simulink library "BatteryPack_192S3P"  (R2025a)
settings: Solver=VariableStepAuto  StartTime=0.0  StopTime=10.0  RelTol=1e-3
undefined symbols (not defined in the file or in its folder): battery_builder_rtmsupport, gcbh
libraries: BatteryPack_192S3P_lib x28, nesl_utility x1, coolingPlateThermal_lib x1, fl_lib x1
(part 3 of 3)

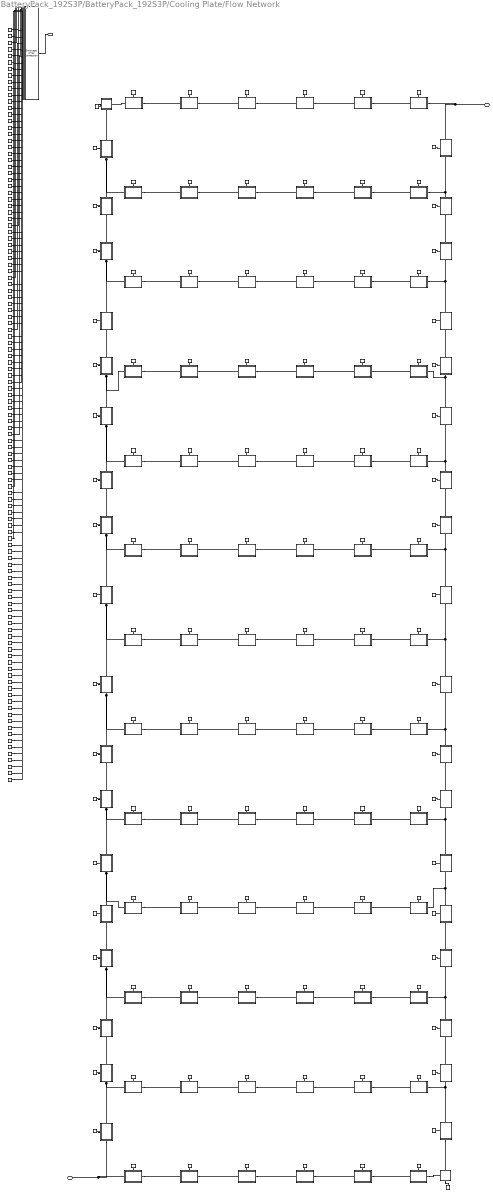
== system BatteryPack_192S3P/BatteryPack_192S3P/Cooling Plate/Flow Network ==
  note: Partition [6,8]
  note: Partition [6,7]
  note: Partition [6,6]
  note: Partition [6,5]
  note: Partition [6,4]
  note: Partition [6,3]
  note: Partition [6,2]
  note: Partition [6,1]
  note: Partition [5,8]
  note: Partition [5,7]
  note: Partition [5,6]
  note: Partition [5,5]
  note: Partition [5,4]
  note: Partition [5,3]
  note: Partition [5,2]
  note: Partition [5,1]
  note: Partition [4,8]
  note: Partition [4,7]
  note: Partition [4,6]
  note: Partition [4,5]
  note: Partition [4,4]
  note: Partition [4,3]
  note: Partition [4,2]
  note: Partition [4,1]
  note: Partition [3,8]
  note: Partition [3,7]
  note: Partition [3,6]
  note: Partition [3,5]
  note: Partition [3,4]
  note: Partition [3,3]
  note: Partition [3,2]
  note: Partition [3,1]
  note: Partition [2,8]
  note: Partition [2,7]
  note: Partition [2,6]
  note: Partition [2,5]
  note: Partition [2,4]
  note: Partition [2,3]
  note: Partition [2,2]
  note: Partition [2,1]
  note: Partition [1,8]
  note: Partition [1,7]
  note: Partition [1,6]
  note: Partition [1,5]
  note: Partition [1,4]
  note: Partition [1,3]
  note: Partition [1,2]
  note: Partition [1,1]
  Array Connection : SimscapeArrayConnection  Domain=foundation.thermal.thermal  NumScalarElements=116
  Bend1_1 : Subsystem  ReferencedSubsystem=BendSubsystemWithMask  lengthPipe=0.0031376  areaPipe=3.1416e-06  diaPipe=0.002  dirPipeOrientBend=up-right
      settings: PortSchema="{\"entries\":[{\"content\":{\"sides\":[{\"content\":{\"connectorIds\":[\"LConn1\"]},\"type\":\"ConnectorPlacement.EquallySpacedRectSide\",\"uuid\":\"064b9882-c01d-4ca6-b21a-bda87b570164\"},{\"content\":{\"side\":\"RIGHT\"},\"type\":\"ConnectorPlacement.EquallySpacedRectSide\",\"uuid\":\"eee751c1-0ee2-4a08-90dc-cac4f5822e04\"},{\"content\":{\"connectorIds\":[\"LConn2\"],\"side\":\"TOP\"},\"type\":\"ConnectorPlacement.EquallySpacedRectSide\",\"uuid\":\"508b7d1b-f548-4587-b0be-a567f0211289\"},{\"content\":{\"connectorIds\":[\"RConn1\"],\"side\":\"BOTTOM\"},\"type\":\"ConnectorPlacement.EquallySpacedRectSide\",\"uuid\":\"316bf1a6-1632-45cd-a339-45482f1cc5f7\"}]},\"type\":\"ConnectorPlacement.EquallySpacedConnector\",\"uuid\":\"7f420bea-eb7e-4a98-ba9c-58ec0a31ea83\"}],\"packageUris\":[\"http://schema.mathworks.com/mf0/Connector/R2020b\"],\"version\":\"1.0\"}"
  Bend2_1 : Subsystem  ReferencedSubsystem=BendSubsystemWithMask  lengthPipe=0.0031376  areaPipe=3.1416e-06  diaPipe=0.002  dirPipeOrientBend=up-right
      settings: PortSchema="{\"entries\":[{\"content\":{\"sides\":[{\"content\":{\"connectorIds\":[\"LConn1\"]},\"type\":\"ConnectorPlacement.EquallySpacedRectSide\",\"uuid\":\"064b9882-c01d-4ca6-b21a-bda87b570164\"},{\"content\":{\"side\":\"RIGHT\"},\"type\":\"ConnectorPlacement.EquallySpacedRectSide\",\"uuid\":\"eee751c1-0ee2-4a08-90dc-cac4f5822e04\"},{\"content\":{\"connectorIds\":[\"LConn2\"],\"side\":\"TOP\"},\"type\":\"ConnectorPlacement.EquallySpacedRectSide\",\"uuid\":\"508b7d1b-f548-4587-b0be-a567f0211289\"},{\"content\":{\"connectorIds\":[\"RConn1\"],\"side\":\"BOTTOM\"},\"type\":\"ConnectorPlacement.EquallySpacedRectSide\",\"uuid\":\"0f8d4577-782b-4a2e-bd78-882efcc560dd\"}]},\"type\":\"ConnectorPlacement.EquallySpacedConnector\",\"uuid\":\"7f420bea-eb7e-4a98-ba9c-58ec0a31ea83\"}],\"packageUris\":[\"http://schema.mathworks.com/mf0/Connector/R2020b\"],\"version\":\"1.0\"}"
  H_10_1 : ConnectionLabel  Label=H_10_1
  H_10_1_bus : ConnectionLabel  Label=H_10_1
  H_10_2 : ConnectionLabel  Label=H_10_2
  H_10_2_bus : ConnectionLabel  Label=H_10_2
  H_10_3 : ConnectionLabel  Label=H_10_3
  H_10_3_bus : ConnectionLabel  Label=H_10_3
  H_10_4 : ConnectionLabel  Label=H_10_4
  H_10_4_bus : ConnectionLabel  Label=H_10_4
  H_10_5 : ConnectionLabel  Label=H_10_5
  H_10_5_bus : ConnectionLabel  Label=H_10_5
  H_10_6 : ConnectionLabel  Label=H_10_6
  H_10_6_bus : ConnectionLabel  Label=H_10_6
  H_11_1 : ConnectionLabel  Label=H_11_1
  H_11_1_bus : ConnectionLabel  Label=H_11_1
  H_11_2 : ConnectionLabel  Label=H_11_2
  H_11_2_bus : ConnectionLabel  Label=H_11_2
  H_11_3 : ConnectionLabel  Label=H_11_3
  H_11_3_bus : ConnectionLabel  Label=H_11_3
  H_11_4 : ConnectionLabel  Label=H_11_4
  H_11_4_bus : ConnectionLabel  Label=H_11_4
  H_11_5 : ConnectionLabel  Label=H_11_5
  H_11_5_bus : ConnectionLabel  Label=H_11_5
  H_11_6 : ConnectionLabel  Label=H_11_6
  H_11_6_bus : ConnectionLabel  Label=H_11_6
  H_12_1 : ConnectionLabel  Label=H_12_1
  H_12_1_bus : ConnectionLabel  Label=H_12_1
  H_12_2 : ConnectionLabel  Label=H_12_2
  H_12_2_bus : ConnectionLabel  Label=H_12_2
  H_12_3 : ConnectionLabel  Label=H_12_3
  H_12_3_bus : ConnectionLabel  Label=H_12_3
  H_12_4 : ConnectionLabel  Label=H_12_4
  H_12_4_bus : ConnectionLabel  Label=H_12_4
  H_12_5 : ConnectionLabel  Label=H_12_5
  H_12_5_bus : ConnectionLabel  Label=H_12_5
  H_12_6 : ConnectionLabel  Label=H_12_6
  H_12_6_bus : ConnectionLabel  Label=H_12_6
  H_13_1 : ConnectionLabel  Label=H_13_1
  H_13_1_bus : ConnectionLabel  Label=H_13_1
  H_13_2 : ConnectionLabel  Label=H_13_2
  H_13_2_bus : ConnectionLabel  Label=H_13_2
  H_13_3 : ConnectionLabel  Label=H_13_3
  H_13_3_bus : ConnectionLabel  Label=H_13_3
  H_13_4 : ConnectionLabel  Label=H_13_4
  H_13_4_bus : ConnectionLabel  Label=H_13_4
  H_13_5 : ConnectionLabel  Label=H_13_5
  H_13_5_bus : ConnectionLabel  Label=H_13_5
  H_13_6 : ConnectionLabel  Label=H_13_6
  H_13_6_bus : ConnectionLabel  Label=H_13_6
  H_14_1 : ConnectionLabel  Label=H_14_1
  H_14_1_bus : ConnectionLabel  Label=H_14_1
  H_15_1 : ConnectionLabel  Label=H_15_1
  H_15_1_bus : ConnectionLabel  Label=H_15_1
  H_15_2 : ConnectionLabel  Label=H_15_2
  H_15_2_bus : ConnectionLabel  Label=H_15_2
  H_16_1 : ConnectionLabel  Label=H_16_1
  H_16_1_bus : ConnectionLabel  Label=H_16_1
  H_16_2 : ConnectionLabel  Label=H_16_2
  H_16_2_bus : ConnectionLabel  Label=H_16_2
  H_17_1 : ConnectionLabel  Label=H_17_1
  H_17_1_bus : ConnectionLabel  Label=H_17_1
  H_18_1 : ConnectionLabel  Label=H_18_1
  H_18_1_bus : ConnectionLabel  Label=H_18_1
  H_18_2 : ConnectionLabel  Label=H_18_2
  H_18_2_bus : ConnectionLabel  Label=H_18_2
  H_19_1 : ConnectionLabel  Label=H_19_1
  H_19_1_bus : ConnectionLabel  Label=H_19_1
  H_1_1 : ConnectionLabel  Label=H_1_1
  H_1_1_bus : ConnectionLabel  Label=H_1_1
  H_1_2 : ConnectionLabel  Label=H_1_2
  H_1_2_bus : ConnectionLabel  Label=H_1_2
  H_1_3 : ConnectionLabel  Label=H_1_3
  H_1_3_bus : ConnectionLabel  Label=H_1_3
  H_1_4 : ConnectionLabel  Label=H_1_4
  H_1_4_bus : ConnectionLabel  Label=H_1_4
  H_1_5 : ConnectionLabel  Label=H_1_5
  H_1_5_bus : ConnectionLabel  Label=H_1_5
  H_1_6 : ConnectionLabel  Label=H_1_6
  H_1_6_bus : ConnectionLabel  Label=H_1_6
  H_20_1 : ConnectionLabel  Label=H_20_1
  H_20_1_bus : ConnectionLabel  Label=H_20_1
  H_21_1 : ConnectionLabel  Label=H_21_1
  H_21_1_bus : ConnectionLabel  Label=H_21_1
  H_21_2 : ConnectionLabel  Label=H_21_2
  H_21_2_bus : ConnectionLabel  Label=H_21_2
  H_22_1 : ConnectionLabel  Label=H_22_1
  H_22_1_bus : ConnectionLabel  Label=H_22_1
  H_23_1 : ConnectionLabel  Label=H_23_1
  H_23_1_bus : ConnectionLabel  Label=H_23_1
  H_23_2 : ConnectionLabel  Label=H_23_2
  H_23_2_bus : ConnectionLabel  Label=H_23_2
  H_24_1 : ConnectionLabel  Label=H_24_1
  H_24_1_bus : ConnectionLabel  Label=H_24_1
  H_24_2 : ConnectionLabel  Label=H_24_2
  H_24_2_bus : ConnectionLabel  Label=H_24_2
  H_25_1 : ConnectionLabel  Label=H_25_1
  H_25_1_bus : ConnectionLabel  Label=H_25_1
  H_26_1 : ConnectionLabel  Label=H_26_1
  H_26_1_bus : ConnectionLabel  Label=H_26_1
  H_27_1 : ConnectionLabel  Label=H_27_1
  H_27_1_bus : ConnectionLabel  Label=H_27_1
  H_27_2 : ConnectionLabel  Label=H_27_2
  H_27_2_bus : ConnectionLabel  Label=H_27_2
  H_28_1 : ConnectionLabel  Label=H_28_1
  H_28_1_bus : ConnectionLabel  Label=H_28_1
  H_28_2 : ConnectionLabel  Label=H_28_2
  H_28_2_bus : ConnectionLabel  Label=H_28_2
  H_29_1 : ConnectionLabel  Label=H_29_1
  H_29_1_bus : ConnectionLabel  Label=H_29_1
  H_2_1 : ConnectionLabel  Label=H_2_1
  H_2_1_bus : ConnectionLabel  Label=H_2_1
  H_2_2 : ConnectionLabel  Label=H_2_2
  H_2_2_bus : ConnectionLabel  Label=H_2_2
  H_2_3 : ConnectionLabel  Label=H_2_3
  H_2_3_bus : ConnectionLabel  Label=H_2_3
  H_2_4 : ConnectionLabel  Label=H_2_4
  H_2_4_bus : ConnectionLabel  Label=H_2_4
  H_2_5 : ConnectionLabel  Label=H_2_5
  H_2_5_bus : ConnectionLabel  Label=H_2_5
  H_2_6 : ConnectionLabel  Label=H_2_6
  H_2_6_bus : ConnectionLabel  Label=H_2_6
  H_30_1 : ConnectionLabel  Label=H_30_1
  H_30_1_bus : ConnectionLabel  Label=H_30_1
  H_30_2 : ConnectionLabel  Label=H_30_2
  H_30_2_bus : ConnectionLabel  Label=H_30_2
  H_31_1 : ConnectionLabel  Label=H_31_1
  H_31_1_bus : ConnectionLabel  Label=H_31_1
  H_32_1 : ConnectionLabel  Label=H_32_1
  H_32_1_bus : ConnectionLabel  Label=H_32_1
  H_33_1 : ConnectionLabel  Label=H_33_1
  H_33_1_bus : ConnectionLabel  Label=H_33_1
  H_33_2 : ConnectionLabel  Label=H_33_2
  H_33_2_bus : ConnectionLabel  Label=H_33_2
  H_34_1 : ConnectionLabel  Label=H_34_1
  H_34_1_bus : ConnectionLabel  Label=H_34_1
  H_35_1 : ConnectionLabel  Label=H_35_1
  H_35_1_bus : ConnectionLabel  Label=H_35_1
  H_35_2 : ConnectionLabel  Label=H_35_2
  H_35_2_bus : ConnectionLabel  Label=H_35_2
  H_36_1 : ConnectionLabel  Label=H_36_1
  H_36_1_bus : ConnectionLabel  Label=H_36_1
  H_36_2 : ConnectionLabel  Label=H_36_2
  H_36_2_bus : ConnectionLabel  Label=H_36_2
  H_37_1 : ConnectionLabel  Label=H_37_1
  H_37_1_bus : ConnectionLabel  Label=H_37_1
  H_38_1 : ConnectionLabel  Label=H_38_1
  H_38_1_bus : ConnectionLabel  Label=H_38_1
  H_39_1 : ConnectionLabel  Label=H_39_1
  H_39_1_bus : ConnectionLabel  Label=H_39_1
  H_3_1 : ConnectionLabel  Label=H_3_1
  H_3_1_bus : ConnectionLabel  Label=H_3_1
  H_3_2 : ConnectionLabel  Label=H_3_2
  H_3_2_bus : ConnectionLabel  Label=H_3_2
  H_3_3 : ConnectionLabel  Label=H_3_3
  H_3_3_bus : ConnectionLabel  Label=H_3_3
  H_3_4 : ConnectionLabel  Label=H_3_4
  H_3_4_bus : ConnectionLabel  Label=H_3_4
  H_3_5 : ConnectionLabel  Label=H_3_5
  H_3_5_bus : ConnectionLabel  Label=H_3_5
  H_3_6 : ConnectionLabel  Label=H_3_6
  H_3_6_bus : ConnectionLabel  Label=H_3_6
  H_4_1 : ConnectionLabel  Label=H_4_1
  H_4_1_bus : ConnectionLabel  Label=H_4_1
  H_4_2 : ConnectionLabel  Label=H_4_2
  H_4_2_bus : ConnectionLabel  Label=H_4_2
  H_4_3 : ConnectionLabel  Label=H_4_3
  H_4_3_bus : ConnectionLabel  Label=H_4_3
  H_4_4 : ConnectionLabel  Label=H_4_4
  H_4_4_bus : ConnectionLabel  Label=H_4_4
  H_4_5 : ConnectionLabel  Label=H_4_5
  H_4_5_bus : ConnectionLabel  Label=H_4_5
  H_4_6 : ConnectionLabel  Label=H_4_6
  H_4_6_bus : ConnectionLabel  Label=H_4_6
  H_5_1 : ConnectionLabel  Label=H_5_1
  H_5_1_bus : ConnectionLabel  Label=H_5_1
  H_5_2 : ConnectionLabel  Label=H_5_2
  H_5_2_bus : ConnectionLabel  Label=H_5_2
  H_5_3 : ConnectionLabel  Label=H_5_3
  H_5_3_bus : ConnectionLabel  Label=H_5_3
  H_5_4 : ConnectionLabel  Label=H_5_4
  H_5_4_bus : ConnectionLabel  Label=H_5_4
  H_5_5 : ConnectionLabel  Label=H_5_5
  H_5_5_bus : ConnectionLabel  Label=H_5_5
  H_5_6 : ConnectionLabel  Label=H_5_6
  H_5_6_bus : ConnectionLabel  Label=H_5_6
  H_6_1 : ConnectionLabel  Label=H_6_1
  H_6_1_bus : ConnectionLabel  Label=H_6_1
  H_6_2 : ConnectionLabel  Label=H_6_2
  H_6_2_bus : ConnectionLabel  Label=H_6_2
  H_6_3 : ConnectionLabel  Label=H_6_3
  H_6_3_bus : ConnectionLabel  Label=H_6_3
  H_6_4 : ConnectionLabel  Label=H_6_4
  H_6_4_bus : ConnectionLabel  Label=H_6_4
  H_6_5 : ConnectionLabel  Label=H_6_5
  H_6_5_bus : ConnectionLabel  Label=H_6_5
  H_6_6 : ConnectionLabel  Label=H_6_6
  H_6_6_bus : ConnectionLabel  Label=H_6_6
  H_7_1 : ConnectionLabel  Label=H_7_1
  H_7_1_bus : ConnectionLabel  Label=H_7_1
  H_7_2 : ConnectionLabel  Label=H_7_2
  H_7_2_bus : ConnectionLabel  Label=H_7_2
  H_7_3 : ConnectionLabel  Label=H_7_3
  H_7_3_bus : ConnectionLabel  Label=H_7_3
  H_7_4 : ConnectionLabel  Label=H_7_4
  H_7_4_bus : ConnectionLabel  Label=H_7_4
  H_7_5 : ConnectionLabel  Label=H_7_5
  H_7_5_bus : ConnectionLabel  Label=H_7_5
  H_7_6 : ConnectionLabel  Label=H_7_6
  H_7_6_bus : ConnectionLabel  Label=H_7_6
  H_8_1 : ConnectionLabel  Label=H_8_1
  H_8_1_bus : ConnectionLabel  Label=H_8_1
  H_8_2 : ConnectionLabel  Label=H_8_2
  H_8_2_bus : ConnectionLabel  Label=H_8_2
  H_8_3 : ConnectionLabel  Label=H_8_3
  H_8_3_bus : ConnectionLabel  Label=H_8_3
  H_8_4 : ConnectionLabel  Label=H_8_4
  H_8_4_bus : ConnectionLabel  Label=H_8_4
  H_8_5 : ConnectionLabel  Label=H_8_5
  H_8_5_bus : ConnectionLabel  Label=H_8_5
  H_8_6 : ConnectionLabel  Label=H_8_6
  H_8_6_bus : ConnectionLabel  Label=H_8_6
  H_9_1 : ConnectionLabel  Label=H_9_1
  H_9_1_bus : ConnectionLabel  Label=H_9_1
  H_9_2 : ConnectionLabel  Label=H_9_2
  H_9_2_bus : ConnectionLabel  Label=H_9_2
  H_9_3 : ConnectionLabel  Label=H_9_3
  H_9_3_bus : ConnectionLabel  Label=H_9_3
  H_9_4 : ConnectionLabel  Label=H_9_4
  H_9_4_bus : ConnectionLabel  Label=H_9_4
  H_9_5 : ConnectionLabel  Label=H_9_5
  H_9_5_bus : ConnectionLabel  Label=H_9_5
  H_9_6 : ConnectionLabel  Label=H_9_6
  H_9_6_bus : ConnectionLabel  Label=H_9_6
  Pipe10_1 : Subsystem  ReferencedSubsystem=PipeSubsystemWithMask  lengthPipe=0.35833  areaPipe=3.1416e-06  diaPipe=0.002  directionPipe=right
      settings: PortSchema="{\"entries\":[{\"content\":{\"sides\":[{\"content\":{\"connectorIds\":[\"LConn1\"]},\"type\":\"ConnectorPlacement.EquallySpacedRectSide\",\"uuid\":\"064b9882-c01d-4ca6-b21a-bda87b570164\"},{\"content\":{\"connectorIds\":[\"RConn1\"],\"side\":\"RIGHT\"},\"type\":\"ConnectorPlacement.EquallySpacedRectSide\",\"uuid\":\"eee751c1-0ee2-4a08-90dc-cac4f5822e04\"},{\"content\":{\"connectorIds\":[\"LConn2\"],\"side\":\"TOP\"},\"type\":\"ConnectorPlacement.EquallySpacedRectSide\",\"uuid\":\"508b7d1b-f548-4587-b0be-a567f0211289\"}]},\"type\":\"ConnectorPlacement.EquallySpacedConnector\",\"uuid\":\"7f420bea-eb7e-4a98-ba9c-58ec0a31ea83\"}],\"packageUris\":[\"http://schema.mathworks.com/mf0/Connector/R2020b\"],\"version\":\"1.0\"}"
  Pipe10_{2..5} (4 alike) : Subsystem  ReferencedSubsystem=PipeSubsystemWithMask  lengthPipe=0.38333  areaPipe=3.1416e-06  diaPipe=0.002  directionPipe=right
      settings: PortSchema="{\"entries\":[{\"content\":{\"sides\":[{\"content\":{\"connectorIds\":[\"LConn1\"]},\"type\":\"ConnectorPlacement.EquallySpacedRectSide\",\"uuid\":\"064b9882-c01d-4ca6-b21a-bda87b570164\"},{\"content\":{\"connectorIds\":[\"RConn1\"],\"side\":\"RIGHT\"},\"type\":\"ConnectorPlacement.EquallySpacedRectSide\",\"uuid\":\"eee751c1-0ee2-4a08-90dc-cac4f5822e04\"},{\"content\":{\"connectorIds\":[\"LConn2\"],\"side\":\"TOP\"},\"type\":\"ConnectorPlacement.EquallySpacedRectSide\",\"uuid\":\"508b7d1b-f548-4587-b0be-a567f0211289\"}]},\"type\":\"ConnectorPlacement.EquallySpacedConnector\",\"uuid\":\"7f420bea-eb7e-4a98-ba9c-58ec0a31ea83\"}],\"packageUris\":[\"http://schema.mathworks.com/mf0/Connector/R2020b\"],\"version\":\"1.0\"}"
  Pipe10_6 : Subsystem  ReferencedSubsystem=PipeSubsystemWithMask  lengthPipe=0.35833  areaPipe=3.1416e-06  diaPipe=0.002  directionPipe=right
      settings: PortSchema="{\"entries\":[{\"content\":{\"sides\":[{\"content\":{\"connectorIds\":[\"LConn1\"]},\"type\":\"ConnectorPlacement.EquallySpacedRectSide\",\"uuid\":\"064b9882-c01d-4ca6-b21a-bda87b570164\"},{\"content\":{\"connectorIds\":[\"RConn1\"],\"side\":\"RIGHT\"},\"type\":\"ConnectorPlacement.EquallySpacedRectSide\",\"uuid\":\"eee751c1-0ee2-4a08-90dc-cac4f5822e04\"},{\"content\":{\"connectorIds\":[\"LConn2\"],\"side\":\"TOP\"},\"type\":\"ConnectorPlacement.EquallySpacedRectSide\",\"uuid\":\"508b7d1b-f548-4587-b0be-a567f0211289\"}]},\"type\":\"ConnectorPlacement.EquallySpacedConnector\",\"uuid\":\"7f420bea-eb7e-4a98-ba9c-58ec0a31ea83\"}],\"packageUris\":[\"http://schema.mathworks.com/mf0/Connector/R2020b\"],\"version\":\"1.0\"}"
  Pipe11_1 : Subsystem  ReferencedSubsystem=PipeSubsystemWithMask  lengthPipe=0.35833  areaPipe=3.1416e-06  diaPipe=0.002  directionPipe=right
      settings: PortSchema="{\"entries\":[{\"content\":{\"sides\":[{\"content\":{\"connectorIds\":[\"LConn1\"]},\"type\":\"ConnectorPlacement.EquallySpacedRectSide\",\"uuid\":\"064b9882-c01d-4ca6-b21a-bda87b570164\"},{\"content\":{\"connectorIds\":[\"RConn1\"],\"side\":\"RIGHT\"},\"type\":\"ConnectorPlacement.EquallySpacedRectSide\",\"uuid\":\"eee751c1-0ee2-4a08-90dc-cac4f5822e04\"},{\"content\":{\"connectorIds\":[\"LConn2\"],\"side\":\"TOP\"},\"type\":\"ConnectorPlacement.EquallySpacedRectSide\",\"uuid\":\"508b7d1b-f548-4587-b0be-a567f0211289\"}]},\"type\":\"ConnectorPlacement.EquallySpacedConnector\",\"uuid\":\"7f420bea-eb7e-4a98-ba9c-58ec0a31ea83\"}],\"packageUris\":[\"http://schema.mathworks.com/mf0/Connector/R2020b\"],\"version\":\"1.0\"}"
  Pipe11_{2..5} (4 alike) : Subsystem  ReferencedSubsystem=PipeSubsystemWithMask  lengthPipe=0.38333  areaPipe=3.1416e-06  diaPipe=0.002  directionPipe=right
      settings: PortSchema="{\"entries\":[{\"content\":{\"sides\":[{\"content\":{\"connectorIds\":[\"LConn1\"]},\"type\":\"ConnectorPlacement.EquallySpacedRectSide\",\"uuid\":\"064b9882-c01d-4ca6-b21a-bda87b570164\"},{\"content\":{\"connectorIds\":[\"RConn1\"],\"side\":\"RIGHT\"},\"type\":\"ConnectorPlacement.EquallySpacedRectSide\",\"uuid\":\"eee751c1-0ee2-4a08-90dc-cac4f5822e04\"},{\"content\":{\"connectorIds\":[\"LConn2\"],\"side\":\"TOP\"},\"type\":\"ConnectorPlacement.EquallySpacedRectSide\",\"uuid\":\"508b7d1b-f548-4587-b0be-a567f0211289\"}]},\"type\":\"ConnectorPlacement.EquallySpacedConnector\",\"uuid\":\"7f420bea-eb7e-4a98-ba9c-58ec0a31ea83\"}],\"packageUris\":[\"http://schema.mathworks.com/mf0/Connector/R2020b\"],\"version\":\"1.0\"}"
  Pipe11_6 : Subsystem  ReferencedSubsystem=PipeSubsystemWithMask  lengthPipe=0.35833  areaPipe=3.1416e-06  diaPipe=0.002  directionPipe=right
      settings: PortSchema="{\"entries\":[{\"content\":{\"sides\":[{\"content\":{\"connectorIds\":[\"LConn1\"]},\"type\":\"ConnectorPlacement.EquallySpacedRectSide\",\"uuid\":\"064b9882-c01d-4ca6-b21a-bda87b570164\"},{\"content\":{\"connectorIds\":[\"RConn1\"],\"side\":\"RIGHT\"},\"type\":\"ConnectorPlacement.EquallySpacedRectSide\",\"uuid\":\"eee751c1-0ee2-4a08-90dc-cac4f5822e04\"},{\"content\":{\"connectorIds\":[\"LConn2\"],\"side\":\"TOP\"},\"type\":\"ConnectorPlacement.EquallySpacedRectSide\",\"uuid\":\"508b7d1b-f548-4587-b0be-a567f0211289\"}]},\"type\":\"ConnectorPlacement.EquallySpacedConnector\",\"uuid\":\"7f420bea-eb7e-4a98-ba9c-58ec0a31ea83\"}],\"packageUris\":[\"http://schema.mathworks.com/mf0/Connector/R2020b\"],\"version\":\"1.0\"}"
  Pipe12_1 : Subsystem  ReferencedSubsystem=PipeSubsystemWithMask  lengthPipe=0.35833  areaPipe=3.1416e-06  diaPipe=0.002  directionPipe=right
      settings: PortSchema="{\"entries\":[{\"content\":{\"sides\":[{\"content\":{\"connectorIds\":[\"LConn1\"]},\"type\":\"ConnectorPlacement.EquallySpacedRectSide\",\"uuid\":\"064b9882-c01d-4ca6-b21a-bda87b570164\"},{\"content\":{\"connectorIds\":[\"RConn1\"],\"side\":\"RIGHT\"},\"type\":\"ConnectorPlacement.EquallySpacedRectSide\",\"uuid\":\"eee751c1-0ee2-4a08-90dc-cac4f5822e04\"},{\"content\":{\"connectorIds\":[\"LConn2\"],\"side\":\"TOP\"},\"type\":\"ConnectorPlacement.EquallySpacedRectSide\",\"uuid\":\"508b7d1b-f548-4587-b0be-a567f0211289\"}]},\"type\":\"ConnectorPlacement.EquallySpacedConnector\",\"uuid\":\"7f420bea-eb7e-4a98-ba9c-58ec0a31ea83\"}],\"packageUris\":[\"http://schema.mathworks.com/mf0/Connector/R2020b\"],\"version\":\"1.0\"}"
  Pipe12_{2..5} (4 alike) : Subsystem  ReferencedSubsystem=PipeSubsystemWithMask  lengthPipe=0.38333  areaPipe=3.1416e-06  diaPipe=0.002  directionPipe=right
      settings: PortSchema="{\"entries\":[{\"content\":{\"sides\":[{\"content\":{\"connectorIds\":[\"LConn1\"]},\"type\":\"ConnectorPlacement.EquallySpacedRectSide\",\"uuid\":\"064b9882-c01d-4ca6-b21a-bda87b570164\"},{\"content\":{\"connectorIds\":[\"RConn1\"],\"side\":\"RIGHT\"},\"type\":\"ConnectorPlacement.EquallySpacedRectSide\",\"uuid\":\"eee751c1-0ee2-4a08-90dc-cac4f5822e04\"},{\"content\":{\"connectorIds\":[\"LConn2\"],\"side\":\"TOP\"},\"type\":\"ConnectorPlacement.EquallySpacedRectSide\",\"uuid\":\"508b7d1b-f548-4587-b0be-a567f0211289\"}]},\"type\":\"ConnectorPlacement.EquallySpacedConnector\",\"uuid\":\"7f420bea-eb7e-4a98-ba9c-58ec0a31ea83\"}],\"packageUris\":[\"http://schema.mathworks.com/mf0/Connector/R2020b\"],\"version\":\"1.0\"}"
  Pipe12_6 : Subsystem  ReferencedSubsystem=PipeSubsystemWithMask  lengthPipe=0.35833  areaPipe=3.1416e-06  diaPipe=0.002  directionPipe=right
      settings: PortSchema="{\"entries\":[{\"content\":{\"sides\":[{\"content\":{\"connectorIds\":[\"LConn1\"]},\"type\":\"ConnectorPlacement.EquallySpacedRectSide\",\"uuid\":\"064b9882-c01d-4ca6-b21a-bda87b570164\"},{\"content\":{\"connectorIds\":[\"RConn1\"],\"side\":\"RIGHT\"},\"type\":\"ConnectorPlacement.EquallySpacedRectSide\",\"uuid\":\"eee751c1-0ee2-4a08-90dc-cac4f5822e04\"},{\"content\":{\"connectorIds\":[\"LConn2\"],\"side\":\"TOP\"},\"type\":\"ConnectorPlacement.EquallySpacedRectSide\",\"uuid\":\"508b7d1b-f548-4587-b0be-a567f0211289\"}]},\"type\":\"ConnectorPlacement.EquallySpacedConnector\",\"uuid\":\"7f420bea-eb7e-4a98-ba9c-58ec0a31ea83\"}],\"packageUris\":[\"http://schema.mathworks.com/mf0/Connector/R2020b\"],\"version\":\"1.0\"}"
  Pipe13_1 : Subsystem  ReferencedSubsystem=PipeSubsystemWithMask  lengthPipe=0.35633  areaPipe=3.1416e-06  diaPipe=0.002  directionPipe=right
      settings: PortSchema="{\"entries\":[{\"content\":{\"sides\":[{\"content\":{\"connectorIds\":[\"LConn1\"]},\"type\":\"ConnectorPlacement.EquallySpacedRectSide\",\"uuid\":\"064b9882-c01d-4ca6-b21a-bda87b570164\"},{\"content\":{\"connectorIds\":[\"RConn1\"],\"side\":\"RIGHT\"},\"type\":\"ConnectorPlacement.EquallySpacedRectSide\",\"uuid\":\"eee751c1-0ee2-4a08-90dc-cac4f5822e04\"},{\"content\":{\"connectorIds\":[\"LConn2\"],\"side\":\"TOP\"},\"type\":\"ConnectorPlacement.EquallySpacedRectSide\",\"uuid\":\"508b7d1b-f548-4587-b0be-a567f0211289\"}]},\"type\":\"ConnectorPlacement.EquallySpacedConnector\",\"uuid\":\"7f420bea-eb7e-4a98-ba9c-58ec0a31ea83\"}],\"packageUris\":[\"http://schema.mathworks.com/mf0/Connector/R2020b\"],\"version\":\"1.0\"}"
  Pipe13_{2..5} (4 alike) : Subsystem  ReferencedSubsystem=PipeSubsystemWithMask  lengthPipe=0.38333  areaPipe=3.1416e-06  diaPipe=0.002  directionPipe=right
      settings: PortSchema="{\"entries\":[{\"content\":{\"sides\":[{\"content\":{\"connectorIds\":[\"LConn1\"]},\"type\":\"ConnectorPlacement.EquallySpacedRectSide\",\"uuid\":\"064b9882-c01d-4ca6-b21a-bda87b570164\"},{\"content\":{\"connectorIds\":[\"RConn1\"],\"side\":\"RIGHT\"},\"type\":\"ConnectorPlacement.EquallySpacedRectSide\",\"uuid\":\"eee751c1-0ee2-4a08-90dc-cac4f5822e04\"},{\"content\":{\"connectorIds\":[\"LConn2\"],\"side\":\"TOP\"},\"type\":\"ConnectorPlacement.EquallySpacedRectSide\",\"uuid\":\"508b7d1b-f548-4587-b0be-a567f0211289\"}]},\"type\":\"ConnectorPlacement.EquallySpacedConnector\",\"uuid\":\"7f420bea-eb7e-4a98-ba9c-58ec0a31ea83\"}],\"packageUris\":[\"http://schema.mathworks.com/mf0/Connector/R2020b\"],\"version\":\"1.0\"}"
  Pipe13_6 : Subsystem  ReferencedSubsystem=PipeSubsystemWithMask  lengthPipe=0.35833  areaPipe=3.1416e-06  diaPipe=0.002  directionPipe=right
      settings: PortSchema="{\"entries\":[{\"content\":{\"sides\":[{\"content\":{\"connectorIds\":[\"LConn1\"]},\"type\":\"ConnectorPlacement.EquallySpacedRectSide\",\"uuid\":\"064b9882-c01d-4ca6-b21a-bda87b570164\"},{\"content\":{\"connectorIds\":[\"RConn1\"],\"side\":\"RIGHT\"},\"type\":\"ConnectorPlacement.EquallySpacedRectSide\",\"uuid\":\"eee751c1-0ee2-4a08-90dc-cac4f5822e04\"},{\"content\":{\"connectorIds\":[\"LConn2\"],\"side\":\"TOP\"},\"type\":\"ConnectorPlacement.EquallySpacedRectSide\",\"uuid\":\"508b7d1b-f548-4587-b0be-a567f0211289\"}]},\"type\":\"ConnectorPlacement.EquallySpacedConnector\",\"uuid\":\"7f420bea-eb7e-4a98-ba9c-58ec0a31ea83\"}],\"packageUris\":[\"http://schema.mathworks.com/mf0/Connector/R2020b\"],\"version\":\"1.0\"}"
  Pipe14_1 : Subsystem  ReferencedSubsystem=PipeSubsystemWithMask  lengthPipe=0.1  areaPipe=3.1416e-06  diaPipe=0.002  directionPipe=up
      settings: PortSchema="{\"entries\":[{\"content\":{\"sides\":[{\"content\":{\"connectorIds\":[\"LConn1\"]},\"type\":\"ConnectorPlacement.EquallySpacedRectSide\",\"uuid\":\"064b9882-c01d-4ca6-b21a-bda87b570164\"},{\"content\":{\"connectorIds\":[\"RConn1\"],\"side\":\"RIGHT\"},\"type\":\"ConnectorPlacement.EquallySpacedRectSide\",\"uuid\":\"eee751c1-0ee2-4a08-90dc-cac4f5822e04\"},{\"content\":{\"connectorIds\":[\"LConn2\"],\"side\":\"TOP\"},\"type\":\"ConnectorPlacement.EquallySpacedRectSide\",\"uuid\":\"508b7d1b-f548-4587-b0be-a567f0211289\"}]},\"type\":\"ConnectorPlacement.EquallySpacedConnector\",\"uuid\":\"7f420bea-eb7e-4a98-ba9c-58ec0a31ea83\"}],\"packageUris\":[\"http://schema.mathworks.com/mf0/Connector/R2020b\"],\"version\":\"1.0\"}"
  Pipe15_1 : Subsystem  ReferencedSubsystem=PipeSubsystemWithMask  lengthPipe=0.03125  areaPipe=3.1416e-06  diaPipe=0.002  directionPipe=up
      settings: PortSchema="{\"entries\":[{\"content\":{\"sides\":[{\"content\":{\"connectorIds\":[\"LConn1\"]},\"type\":\"ConnectorPlacement.EquallySpacedRectSide\",\"uuid\":\"064b9882-c01d-4ca6-b21a-bda87b570164\"},{\"content\":{\"connectorIds\":[\"RConn1\"],\"side\":\"RIGHT\"},\"type\":\"ConnectorPlacement.EquallySpacedRectSide\",\"uuid\":\"eee751c1-0ee2-4a08-90dc-cac4f5822e04\"},{\"content\":{\"connectorIds\":[\"LConn2\"],\"side\":\"TOP\"},\"type\":\"ConnectorPlacement.EquallySpacedRectSide\",\"uuid\":\"508b7d1b-f548-4587-b0be-a567f0211289\"}]},\"type\":\"ConnectorPlacement.EquallySpacedConnector\",\"uuid\":\"7f420bea-eb7e-4a98-ba9c-58ec0a31ea83\"}],\"packageUris\":[\"http://schema.mathworks.com/mf0/Connector/R2020b\"],\"version\":\"1.0\"}"
  Pipe15_2 : Subsystem  ReferencedSubsystem=PipeSubsystemWithMask  lengthPipe=0.06875  areaPipe=3.1416e-06  diaPipe=0.002  directionPipe=up
      settings: PortSchema="{\"entries\":[{\"content\":{\"sides\":[{\"content\":{\"connectorIds\":[\"LConn1\"]},\"type\":\"ConnectorPlacement.EquallySpacedRectSide\",\"uuid\":\"064b9882-c01d-4ca6-b21a-bda87b570164\"},{\"content\":{\"connectorIds\":[\"RConn1\"],\"side\":\"RIGHT\"},\"type\":\"ConnectorPlacement.EquallySpacedRectSide\",\"uuid\":\"eee751c1-0ee2-4a08-90dc-cac4f5822e04\"},{\"content\":{\"connectorIds\":[\"LConn2\"],\"side\":\"TOP\"},\"type\":\"ConnectorPlacement.EquallySpacedRectSide\",\"uuid\":\"508b7d1b-f548-4587-b0be-a567f0211289\"}]},\"type\":\"ConnectorPlacement.EquallySpacedConnector\",\"uuid\":\"7f420bea-eb7e-4a98-ba9c-58ec0a31ea83\"}],\"packageUris\":[\"http://schema.mathworks.com/mf0/Connector/R2020b\"],\"version\":\"1.0\"}"
  Pipe16_1 : Subsystem  ReferencedSubsystem=PipeSubsystemWithMask  lengthPipe=0.0875  areaPipe=3.1416e-06  diaPipe=0.002  directionPipe=up
      settings: PortSchema="{\"entries\":[{\"content\":{\"sides\":[{\"content\":{\"connectorIds\":[\"LConn1\"]},\"type\":\"ConnectorPlacement.EquallySpacedRectSide\",\"uuid\":\"064b9882-c01d-4ca6-b21a-bda87b570164\"},{\"content\":{\"connectorIds\":[\"RConn1\"],\"side\":\"RIGHT\"},\"type\":\"ConnectorPlacement.EquallySpacedRectSide\",\"uuid\":\"eee751c1-0ee2-4a08-90dc-cac4f5822e04\"},{\"content\":{\"connectorIds\":[\"LConn2\"],\"side\":\"TOP\"},\"type\":\"ConnectorPlacement.EquallySpacedRectSide\",\"uuid\":\"508b7d1b-f548-4587-b0be-a567f0211289\"}]},\"type\":\"ConnectorPlacement.EquallySpacedConnector\",\"uuid\":\"7f420bea-eb7e-4a98-ba9c-58ec0a31ea83\"}],\"packageUris\":[\"http://schema.mathworks.com/mf0/Connector/R2020b\"],\"version\":\"1.0\"}"
  Pipe16_2 : Subsystem  ReferencedSubsystem=PipeSubsystemWithMask  lengthPipe=0.0125  areaPipe=3.1416e-06  diaPipe=0.002  directionPipe=up
      settings: PortSchema="{\"entries\":[{\"content\":{\"sides\":[{\"content\":{\"connectorIds\":[\"LConn1\"]},\"type\":\"ConnectorPlacement.EquallySpacedRectSide\",\"uuid\":\"064b9882-c01d-4ca6-b21a-bda87b570164\"},{\"content\":{\"connectorIds\":[\"RConn1\"],\"side\":\"RIGHT\"},\"type\":\"ConnectorPlacement.EquallySpacedRectSide\",\"uuid\":\"eee751c1-0ee2-4a08-90dc-cac4f5822e04\"},{\"content\":{\"connectorIds\":[\"LConn2\"],\"side\":\"TOP\"},\"type\":\"ConnectorPlacement.EquallySpacedRectSide\",\"uuid\":\"508b7d1b-f548-4587-b0be-a567f0211289\"}]},\"type\":\"ConnectorPlacement.EquallySpacedConnector\",\"uuid\":\"7f420bea-eb7e-4a98-ba9c-58ec0a31ea83\"}],\"packageUris\":[\"http://schema.mathworks.com/mf0/Connector/R2020b\"],\"version\":\"1.0\"}"
  Pipe17_1 : Subsystem  ReferencedSubsystem=PipeSubsystemWithMask  lengthPipe=0.1  areaPipe=3.1416e-06  diaPipe=0.002  directionPipe=up
      settings: PortSchema="{\"entries\":[{\"content\":{\"sides\":[{\"content\":{\"connectorIds\":[\"LConn1\"]},\"type\":\"ConnectorPlacement.EquallySpacedRectSide\",\"uuid\":\"064b9882-c01d-4ca6-b21a-bda87b570164\"},{\"content\":{\"connectorIds\":[\"RConn1\"],\"side\":\"RIGHT\"},\"type\":\"ConnectorPlacement.EquallySpacedRectSide\",\"uuid\":\"eee751c1-0ee2-4a08-90dc-cac4f5822e04\"},{\"content\":{\"connectorIds\":[\"LConn2\"],\"side\":\"TOP\"},\"type\":\"ConnectorPlacement.EquallySpacedRectSide\",\"uuid\":\"508b7d1b-f548-4587-b0be-a567f0211289\"}]},\"type\":\"ConnectorPlacement.EquallySpacedConnector\",\"uuid\":\"7f420bea-eb7e-4a98-ba9c-58ec0a31ea83\"}],\"packageUris\":[\"http://schema.mathworks.com/mf0/Connector/R2020b\"],\"version\":\"1.0\"}"
  Pipe18_1 : Subsystem  ReferencedSubsystem=PipeSubsystemWithMask  lengthPipe=0.04375  areaPipe=3.1416e-06  diaPipe=0.002  directionPipe=up
      settings: PortSchema="{\"entries\":[{\"content\":{\"sides\":[{\"content\":{\"connectorIds\":[\"LConn1\"]},\"type\":\"ConnectorPlacement.EquallySpacedRectSide\",\"uuid\":\"064b9882-c01d-4ca6-b21a-bda87b570164\"},{\"content\":{\"connectorIds\":[\"RConn1\"],\"side\":\"RIGHT\"},\"type\":\"ConnectorPlacement.EquallySpacedRectSide\",\"uuid\":\"eee751c1-0ee2-4a08-90dc-cac4f5822e04\"},{\"content\":{\"connectorIds\":[\"LConn2\"],\"side\":\"TOP\"},\"type\":\"ConnectorPlacement.EquallySpacedRectSide\",\"uuid\":\"508b7d1b-f548-4587-b0be-a567f0211289\"}]},\"type\":\"ConnectorPlacement.EquallySpacedConnector\",\"uuid\":\"7f420bea-eb7e-4a98-ba9c-58ec0a31ea83\"}],\"packageUris\":[\"http://schema.mathworks.com/mf0/Connector/R2020b\"],\"version\":\"1.0\"}"
  Pipe18_2 : Subsystem  ReferencedSubsystem=PipeSubsystemWithMask  lengthPipe=0.05625  areaPipe=3.1416e-06  diaPipe=0.002  directionPipe=up
      settings: PortSchema="{\"entries\":[{\"content\":{\"sides\":[{\"content\":{\"connectorIds\":[\"LConn1\"]},\"type\":\"ConnectorPlacement.EquallySpacedRectSide\",\"uuid\":\"064b9882-c01d-4ca6-b21a-bda87b570164\"},{\"content\":{\"connectorIds\":[\"RConn1\"],\"side\":\"RIGHT\"},\"type\":\"ConnectorPlacement.EquallySpacedRectSide\",\"uuid\":\"eee751c1-0ee2-4a08-90dc-cac4f5822e04\"},{\"content\":{\"connectorIds\":[\"LConn2\"],\"side\":\"TOP\"},\"type\":\"ConnectorPlacement.EquallySpacedRectSide\",\"uuid\":\"508b7d1b-f548-4587-b0be-a567f0211289\"}]},\"type\":\"ConnectorPlacement.EquallySpacedConnector\",\"uuid\":\"7f420bea-eb7e-4a98-ba9c-58ec0a31ea83\"}],\"packageUris\":[\"http://schema.mathworks.com/mf0/Connector/R2020b\"],\"version\":\"1.0\"}"
  Pipe19_1 : Subsystem  ReferencedSubsystem=PipeSubsystemWithMask  lengthPipe=0.1  areaPipe=3.1416e-06  diaPipe=0.002  directionPipe=up
      settings: PortSchema="{\"entries\":[{\"content\":{\"sides\":[{\"content\":{\"connectorIds\":[\"LConn1\"]},\"type\":\"ConnectorPlacement.EquallySpacedRectSide\",\"uuid\":\"064b9882-c01d-4ca6-b21a-bda87b570164\"},{\"content\":{\"connectorIds\":[\"RConn1\"],\"side\":\"RIGHT\"},\"type\":\"ConnectorPlacement.EquallySpacedRectSide\",\"uuid\":\"eee751c1-0ee2-4a08-90dc-cac4f5822e04\"},{\"content\":{\"connectorIds\":[\"LConn2\"],\"side\":\"TOP\"},\"type\":\"ConnectorPlacement.EquallySpacedRectSide\",\"uuid\":\"508b7d1b-f548-4587-b0be-a567f0211289\"}]},\"type\":\"ConnectorPlacement.EquallySpacedConnector\",\"uuid\":\"7f420bea-eb7e-4a98-ba9c-58ec0a31ea83\"}],\"packageUris\":[\"http://schema.mathworks.com/mf0/Connector/R2020b\"],\"version\":\"1.0\"}"
  Pipe1_1 : Subsystem  ReferencedSubsystem=PipeSubsystemWithMask  lengthPipe=0.35833  areaPipe=3.1416e-06  diaPipe=0.002  directionPipe=right
      settings: PortSchema="{\"entries\":[{\"content\":{\"sides\":[{\"content\":{\"connectorIds\":[\"LConn1\"]},\"type\":\"ConnectorPlacement.EquallySpacedRectSide\",\"uuid\":\"064b9882-c01d-4ca6-b21a-bda87b570164\"},{\"content\":{\"connectorIds\":[\"RConn1\"],\"side\":\"RIGHT\"},\"type\":\"ConnectorPlacement.EquallySpacedRectSide\",\"uuid\":\"eee751c1-0ee2-4a08-90dc-cac4f5822e04\"},{\"content\":{\"connectorIds\":[\"LConn2\"],\"side\":\"TOP\"},\"type\":\"ConnectorPlacement.EquallySpacedRectSide\",\"uuid\":\"508b7d1b-f548-4587-b0be-a567f0211289\"}]},\"type\":\"ConnectorPlacement.EquallySpacedConnector\",\"uuid\":\"7f420bea-eb7e-4a98-ba9c-58ec0a31ea83\"}],\"packageUris\":[\"http://schema.mathworks.com/mf0/Connector/R2020b\"],\"version\":\"1.0\"}"
  Pipe1_{2..5} (4 alike) : Subsystem  ReferencedSubsystem=PipeSubsystemWithMask  lengthPipe=0.38333  areaPipe=3.1416e-06  diaPipe=0.002  directionPipe=right
      settings: PortSchema="{\"entries\":[{\"content\":{\"sides\":[{\"content\":{\"connectorIds\":[\"LConn1\"]},\"type\":\"ConnectorPlacement.EquallySpacedRectSide\",\"uuid\":\"064b9882-c01d-4ca6-b21a-bda87b570164\"},{\"content\":{\"connectorIds\":[\"RConn1\"],\"side\":\"RIGHT\"},\"type\":\"ConnectorPlacement.EquallySpacedRectSide\",\"uuid\":\"eee751c1-0ee2-4a08-90dc-cac4f5822e04\"},{\"content\":{\"connectorIds\":[\"LConn2\"],\"side\":\"TOP\"},\"type\":\"ConnectorPlacement.EquallySpacedRectSide\",\"uuid\":\"508b7d1b-f548-4587-b0be-a567f0211289\"}]},\"type\":\"ConnectorPlacement.EquallySpacedConnector\",\"uuid\":\"7f420bea-eb7e-4a98-ba9c-58ec0a31ea83\"}],\"packageUris\":[\"http://schema.mathworks.com/mf0/Connector/R2020b\"],\"version\":\"1.0\"}"
  Pipe1_6 : Subsystem  ReferencedSubsystem=PipeSubsystemWithMask  lengthPipe=0.35633  areaPipe=3.1416e-06  diaPipe=0.002  directionPipe=right
      settings: PortSchema="{\"entries\":[{\"content\":{\"sides\":[{\"content\":{\"connectorIds\":[\"LConn1\"]},\"type\":\"ConnectorPlacement.EquallySpacedRectSide\",\"uuid\":\"064b9882-c01d-4ca6-b21a-bda87b570164\"},{\"content\":{\"connectorIds\":[\"RConn1\"],\"side\":\"RIGHT\"},\"type\":\"ConnectorPlacement.EquallySpacedRectSide\",\"uuid\":\"eee751c1-0ee2-4a08-90dc-cac4f5822e04\"},{\"content\":{\"connectorIds\":[\"LConn2\"],\"side\":\"TOP\"},\"type\":\"ConnectorPlacement.EquallySpacedRectSide\",\"uuid\":\"508b7d1b-f548-4587-b0be-a567f0211289\"}]},\"type\":\"ConnectorPlacement.EquallySpacedConnector\",\"uuid\":\"7f420bea-eb7e-4a98-ba9c-58ec0a31ea83\"}],\"packageUris\":[\"http://schema.mathworks.com/mf0/Connector/R2020b\"],\"version\":\"1.0\"}"
  Pipe20_1 : Subsystem  ReferencedSubsystem=PipeSubsystemWithMask  lengthPipe=0.1  areaPipe=3.1416e-06  diaPipe=0.002  directionPipe=up
      settings: PortSchema="{\"entries\":[{\"content\":{\"sides\":[{\"content\":{\"connectorIds\":[\"LConn1\"]},\"type\":\"ConnectorPlacement.EquallySpacedRectSide\",\"uuid\":\"064b9882-c01d-4ca6-b21a-bda87b570164\"},{\"content\":{\"connectorIds\":[\"RConn1\"],\"side\":\"RIGHT\"},\"type\":\"ConnectorPlacement.EquallySpacedRectSide\",\"uuid\":\"eee751c1-0ee2-4a08-90dc-cac4f5822e04\"},{\"content\":{\"connectorIds\":[\"LConn2\"],\"side\":\"TOP\"},\"type\":\"ConnectorPlacement.EquallySpacedRectSide\",\"uuid\":\"508b7d1b-f548-4587-b0be-a567f0211289\"}]},\"type\":\"ConnectorPlacement.EquallySpacedConnector\",\"uuid\":\"7f420bea-eb7e-4a98-ba9c-58ec0a31ea83\"}],\"packageUris\":[\"http://schema.mathworks.com/mf0/Connector/R2020b\"],\"version\":\"1.0\"}"
  Pipe21_1 : Subsystem  ReferencedSubsystem=PipeSubsystemWithMask  lengthPipe=0.05625  areaPipe=3.1416e-06  diaPipe=0.002  directionPipe=up
      settings: PortSchema="{\"entries\":[{\"content\":{\"sides\":[{\"content\":{\"connectorIds\":[\"LConn1\"]},\"type\":\"ConnectorPlacement.EquallySpacedRectSide\",\"uuid\":\"064b9882-c01d-4ca6-b21a-bda87b570164\"},{\"content\":{\"connectorIds\":[\"RConn1\"],\"side\":\"RIGHT\"},\"type\":\"ConnectorPlacement.EquallySpacedRectSide\",\"uuid\":\"eee751c1-0ee2-4a08-90dc-cac4f5822e04\"},{\"content\":{\"connectorIds\":[\"LConn2\"],\"side\":\"TOP\"},\"type\":\"ConnectorPlacement.EquallySpacedRectSide\",\"uuid\":\"508b7d1b-f548-4587-b0be-a567f0211289\"}]},\"type\":\"ConnectorPlacement.EquallySpacedConnector\",\"uuid\":\"7f420bea-eb7e-4a98-ba9c-58ec0a31ea83\"}],\"packageUris\":[\"http://schema.mathworks.com/mf0/Connector/R2020b\"],\"version\":\"1.0\"}"
  Pipe21_2 : Subsystem  ReferencedSubsystem=PipeSubsystemWithMask  lengthPipe=0.04375  areaPipe=3.1416e-06  diaPipe=0.002  directionPipe=up
      settings: PortSchema="{\"entries\":[{\"content\":{\"sides\":[{\"content\":{\"connectorIds\":[\"LConn1\"]},\"type\":\"ConnectorPlacement.EquallySpacedRectSide\",\"uuid\":\"064b9882-c01d-4ca6-b21a-bda87b570164\"},{\"content\":{\"connectorIds\":[\"RConn1\"],\"side\":\"RIGHT\"},\"type\":\"ConnectorPlacement.EquallySpacedRectSide\",\"uuid\":\"eee751c1-0ee2-4a08-90dc-cac4f5822e04\"},{\"content\":{\"connectorIds\":[\"LConn2\"],\"side\":\"TOP\"},\"type\":\"ConnectorPlacement.EquallySpacedRectSide\",\"uuid\":\"508b7d1b-f548-4587-b0be-a567f0211289\"}]},\"type\":\"ConnectorPlacement.EquallySpacedConnector\",\"uuid\":\"7f420bea-eb7e-4a98-ba9c-58ec0a31ea83\"}],\"packageUris\":[\"http://schema.mathworks.com/mf0/Connector/R2020b\"],\"version\":\"1.0\"}"
  Pipe22_1 : Subsystem  ReferencedSubsystem=PipeSubsystemWithMask  lengthPipe=0.1  areaPipe=3.1416e-06  diaPipe=0.002  directionPipe=up
      settings: PortSchema="{\"entries\":[{\"content\":{\"sides\":[{\"content\":{\"connectorIds\":[\"LConn1\"]},\"type\":\"ConnectorPlacement.EquallySpacedRectSide\",\"uuid\":\"064b9882-c01d-4ca6-b21a-bda87b570164\"},{\"content\":{\"connectorIds\":[\"RConn1\"],\"side\":\"RIGHT\"},\"type\":\"ConnectorPlacement.EquallySpacedRectSide\",\"uuid\":\"eee751c1-0ee2-4a08-90dc-cac4f5822e04\"},{\"content\":{\"connectorIds\":[\"LConn2\"],\"side\":\"TOP\"},\"type\":\"ConnectorPlacement.EquallySpacedRectSide\",\"uuid\":\"508b7d1b-f548-4587-b0be-a567f0211289\"}]},\"type\":\"ConnectorPlacement.EquallySpacedConnector\",\"uuid\":\"7f420bea-eb7e-4a98-ba9c-58ec0a31ea83\"}],\"packageUris\":[\"http://schema.mathworks.com/mf0/Connector/R2020b\"],\"version\":\"1.0\"}"
  Pipe23_1 : Subsystem  ReferencedSubsystem=PipeSubsystemWithMask  lengthPipe=0.0125  areaPipe=3.1416e-06  diaPipe=0.002  directionPipe=up
      settings: PortSchema="{\"entries\":[{\"content\":{\"sides\":[{\"content\":{\"connectorIds\":[\"LConn1\"]},\"type\":\"ConnectorPlacement.EquallySpacedRectSide\",\"uuid\":\"064b9882-c01d-4ca6-b21a-bda87b570164\"},{\"content\":{\"connectorIds\":[\"RConn1\"],\"side\":\"RIGHT\"},\"type\":\"ConnectorPlacement.EquallySpacedRectSide\",\"uuid\":\"eee751c1-0ee2-4a08-90dc-cac4f5822e04\"},{\"content\":{\"connectorIds\":[\"LConn2\"],\"side\":\"TOP\"},\"type\":\"ConnectorPlacement.EquallySpacedRectSide\",\"uuid\":\"508b7d1b-f548-4587-b0be-a567f0211289\"}]},\"type\":\"ConnectorPlacement.EquallySpacedConnector\",\"uuid\":\"7f420bea-eb7e-4a98-ba9c-58ec0a31ea83\"}],\"packageUris\":[\"http://schema.mathworks.com/mf0/Connector/R2020b\"],\"version\":\"1.0\"}"
  Pipe23_2 : Subsystem  ReferencedSubsystem=PipeSubsystemWithMask  lengthPipe=0.0875  areaPipe=3.1416e-06  diaPipe=0.002  directionPipe=up
      settings: PortSchema="{\"entries\":[{\"content\":{\"sides\":[{\"content\":{\"connectorIds\":[\"LConn1\"]},\"type\":\"ConnectorPlacement.EquallySpacedRectSide\",\"uuid\":\"064b9882-c01d-4ca6-b21a-bda87b570164\"},{\"content\":{\"connectorIds\":[\"RConn1\"],\"side\":\"RIGHT\"},\"type\":\"ConnectorPlacement.EquallySpacedRectSide\",\"uuid\":\"eee751c1-0ee2-4a08-90dc-cac4f5822e04\"},{\"content\":{\"connectorIds\":[\"LConn2\"],\"side\":\"TOP\"},\"type\":\"ConnectorPlacement.EquallySpacedRectSide\",\"uuid\":\"508b7d1b-f548-4587-b0be-a567f0211289\"}]},\"type\":\"ConnectorPlacement.EquallySpacedConnector\",\"uuid\":\"7f420bea-eb7e-4a98-ba9c-58ec0a31ea83\"}],\"packageUris\":[\"http://schema.mathworks.com/mf0/Connector/R2020b\"],\"version\":\"1.0\"}"
  Pipe24_1 : Subsystem  ReferencedSubsystem=PipeSubsystemWithMask  lengthPipe=0.06875  areaPipe=3.1416e-06  diaPipe=0.002  directionPipe=up
      settings: PortSchema="{\"entries\":[{\"content\":{\"sides\":[{\"content\":{\"connectorIds\":[\"LConn1\"]},\"type\":\"ConnectorPlacement.EquallySpacedRectSide\",\"uuid\":\"064b9882-c01d-4ca6-b21a-bda87b570164\"},{\"content\":{\"connectorIds\":[\"RConn1\"],\"side\":\"RIGHT\"},\"type\":\"ConnectorPlacement.EquallySpacedRectSide\",\"uuid\":\"eee751c1-0ee2-4a08-90dc-cac4f5822e04\"},{\"content\":{\"connectorIds\":[\"LConn2\"],\"side\":\"TOP\"},\"type\":\"ConnectorPlacement.EquallySpacedRectSide\",\"uuid\":\"508b7d1b-f548-4587-b0be-a567f0211289\"}]},\"type\":\"ConnectorPlacement.EquallySpacedConnector\",\"uuid\":\"7f420bea-eb7e-4a98-ba9c-58ec0a31ea83\"}],\"packageUris\":[\"http://schema.mathworks.com/mf0/Connector/R2020b\"],\"version\":\"1.0\"}"
  Pipe24_2 : Subsystem  ReferencedSubsystem=PipeSubsystemWithMask  lengthPipe=0.03125  areaPipe=3.1416e-06  diaPipe=0.002  directionPipe=up
      settings: PortSchema="{\"entries\":[{\"content\":{\"sides\":[{\"content\":{\"connectorIds\":[\"LConn1\"]},\"type\":\"ConnectorPlacement.EquallySpacedRectSide\",\"uuid\":\"064b9882-c01d-4ca6-b21a-bda87b570164\"},{\"content\":{\"connectorIds\":[\"RConn1\"],\"side\":\"RIGHT\"},\"type\":\"ConnectorPlacement.EquallySpacedRectSide\",\"uuid\":\"eee751c1-0ee2-4a08-90dc-cac4f5822e04\"},{\"content\":{\"connectorIds\":[\"LConn2\"],\"side\":\"TOP\"},\"type\":\"ConnectorPlacement.EquallySpacedRectSide\",\"uuid\":\"508b7d1b-f548-4587-b0be-a567f0211289\"}]},\"type\":\"ConnectorPlacement.EquallySpacedConnector\",\"uuid\":\"7f420bea-eb7e-4a98-ba9c-58ec0a31ea83\"}],\"packageUris\":[\"http://schema.mathworks.com/mf0/Connector/R2020b\"],\"version\":\"1.0\"}"
  Pipe25_1 : Subsystem  ReferencedSubsystem=PipeSubsystemWithMask  lengthPipe=0.098  areaPipe=3.1416e-06  diaPipe=0.002  directionPipe=up
      settings: PortSchema="{\"entries\":[{\"content\":{\"sides\":[{\"content\":{\"connectorIds\":[\"LConn1\"]},\"type\":\"ConnectorPlacement.EquallySpacedRectSide\",\"uuid\":\"064b9882-c01d-4ca6-b21a-bda87b570164\"},{\"content\":{\"connectorIds\":[\"RConn1\"],\"side\":\"RIGHT\"},\"type\":\"ConnectorPlacement.EquallySpacedRectSide\",\"uuid\":\"eee751c1-0ee2-4a08-90dc-cac4f5822e04\"},{\"content\":{\"connectorIds\":[\"LConn2\"],\"side\":\"TOP\"},\"type\":\"ConnectorPlacement.EquallySpacedRectSide\",\"uuid\":\"508b7d1b-f548-4587-b0be-a567f0211289\"}]},\"type\":\"ConnectorPlacement.EquallySpacedConnector\",\"uuid\":\"7f420bea-eb7e-4a98-ba9c-58ec0a31ea83\"}],\"packageUris\":[\"http://schema.mathworks.com/mf0/Connector/R2020b\"],\"version\":\"1.0\"}"
  Pipe26_1 : Subsystem  ReferencedSubsystem=PipeSubsystemWithMask  lengthPipe=0.098  areaPipe=3.1416e-06  diaPipe=0.002  directionPipe=up
      settings: PortSchema="{\"entries\":[{\"content\":{\"sides\":[{\"content\":{\"connectorIds\":[\"LConn1\"]},\"type\":\"ConnectorPlacement.EquallySpacedRectSide\",\"uuid\":\"064b9882-c01d-4ca6-b21a-bda87b570164\"},{\"content\":{\"connectorIds\":[\"RConn1\"],\"side\":\"RIGHT\"},\"type\":\"ConnectorPlacement.EquallySpacedRectSide\",\"uuid\":\"eee751c1-0ee2-4a08-90dc-cac4f5822e04\"},{\"content\":{\"connectorIds\":[\"LConn2\"],\"side\":\"TOP\"},\"type\":\"ConnectorPlacement.EquallySpacedRectSide\",\"uuid\":\"508b7d1b-f548-4587-b0be-a567f0211289\"}]},\"type\":\"ConnectorPlacement.EquallySpacedConnector\",\"uuid\":\"7f420bea-eb7e-4a98-ba9c-58ec0a31ea83\"}],\"packageUris\":[\"http://schema.mathworks.com/mf0/Connector/R2020b\"],\"version\":\"1.0\"}"
  Pipe27_1 : Subsystem  ReferencedSubsystem=PipeSubsystemWithMask  lengthPipe=0.03125  areaPipe=3.1416e-06  diaPipe=0.002  directionPipe=up
      settings: PortSchema="{\"entries\":[{\"content\":{\"sides\":[{\"content\":{\"connectorIds\":[\"LConn1\"]},\"type\":\"ConnectorPlacement.EquallySpacedRectSide\",\"uuid\":\"064b9882-c01d-4ca6-b21a-bda87b570164\"},{\"content\":{\"connectorIds\":[\"RConn1\"],\"side\":\"RIGHT\"},\"type\":\"ConnectorPlacement.EquallySpacedRectSide\",\"uuid\":\"eee751c1-0ee2-4a08-90dc-cac4f5822e04\"},{\"content\":{\"connectorIds\":[\"LConn2\"],\"side\":\"TOP\"},\"type\":\"ConnectorPlacement.EquallySpacedRectSide\",\"uuid\":\"508b7d1b-f548-4587-b0be-a567f0211289\"}]},\"type\":\"ConnectorPlacement.EquallySpacedConnector\",\"uuid\":\"7f420bea-eb7e-4a98-ba9c-58ec0a31ea83\"}],\"packageUris\":[\"http://schema.mathworks.com/mf0/Connector/R2020b\"],\"version\":\"1.0\"}"
  Pipe27_2 : Subsystem  ReferencedSubsystem=PipeSubsystemWithMask  lengthPipe=0.06875  areaPipe=3.1416e-06  diaPipe=0.002  directionPipe=up
      settings: PortSchema="{\"entries\":[{\"content\":{\"sides\":[{\"content\":{\"connectorIds\":[\"LConn1\"]},\"type\":\"ConnectorPlacement.EquallySpacedRectSide\",\"uuid\":\"064b9882-c01d-4ca6-b21a-bda87b570164\"},{\"content\":{\"connectorIds\":[\"RConn1\"],\"side\":\"RIGHT\"},\"type\":\"ConnectorPlacement.EquallySpacedRectSide\",\"uuid\":\"eee751c1-0ee2-4a08-90dc-cac4f5822e04\"},{\"content\":{\"connectorIds\":[\"LConn2\"],\"side\":\"TOP\"},\"type\":\"ConnectorPlacement.EquallySpacedRectSide\",\"uuid\":\"508b7d1b-f548-4587-b0be-a567f0211289\"}]},\"type\":\"ConnectorPlacement.EquallySpacedConnector\",\"uuid\":\"7f420bea-eb7e-4a98-ba9c-58ec0a31ea83\"}],\"packageUris\":[\"http://schema.mathworks.com/mf0/Connector/R2020b\"],\"version\":\"1.0\"}"
  Pipe28_1 : Subsystem  ReferencedSubsystem=PipeSubsystemWithMask  lengthPipe=0.0875  areaPipe=3.1416e-06  diaPipe=0.002  directionPipe=up
      settings: PortSchema="{\"entries\":[{\"content\":{\"sides\":[{\"content\":{\"connectorIds\":[\"LConn1\"]},\"type\":\"ConnectorPlacement.EquallySpacedRectSide\",\"uuid\":\"064b9882-c01d-4ca6-b21a-bda87b570164\"},{\"content\":{\"connectorIds\":[\"RConn1\"],\"side\":\"RIGHT\"},\"type\":\"ConnectorPlacement.EquallySpacedRectSide\",\"uuid\":\"eee751c1-0ee2-4a08-90dc-cac4f5822e04\"},{\"content\":{\"connectorIds\":[\"LConn2\"],\"side\":\"TOP\"},\"type\":\"ConnectorPlacement.EquallySpacedRectSide\",\"uuid\":\"508b7d1b-f548-4587-b0be-a567f0211289\"}]},\"type\":\"ConnectorPlacement.EquallySpacedConnector\",\"uuid\":\"7f420bea-eb7e-4a98-ba9c-58ec0a31ea83\"}],\"packageUris\":[\"http://schema.mathworks.com/mf0/Connector/R2020b\"],\"version\":\"1.0\"}"
  Pipe28_2 : Subsystem  ReferencedSubsystem=PipeSubsystemWithMask  lengthPipe=0.0125  areaPipe=3.1416e-06  diaPipe=0.002  directionPipe=up
      settings: PortSchema="{\"entries\":[{\"content\":{\"sides\":[{\"content\":{\"connectorIds\":[\"LConn1\"]},\"type\":\"ConnectorPlacement.EquallySpacedRectSide\",\"uuid\":\"064b9882-c01d-4ca6-b21a-bda87b570164\"},{\"content\":{\"connectorIds\":[\"RConn1\"],\"side\":\"RIGHT\"},\"type\":\"ConnectorPlacement.EquallySpacedRectSide\",\"uuid\":\"eee751c1-0ee2-4a08-90dc-cac4f5822e04\"},{\"content\":{\"connectorIds\":[\"LConn2\"],\"side\":\"TOP\"},\"type\":\"ConnectorPlacement.EquallySpacedRectSide\",\"uuid\":\"508b7d1b-f548-4587-b0be-a567f0211289\"}]},\"type\":\"ConnectorPlacement.EquallySpacedConnector\",\"uuid\":\"7f420bea-eb7e-4a98-ba9c-58ec0a31ea83\"}],\"packageUris\":[\"http://schema.mathworks.com/mf0/Connector/R2020b\"],\"version\":\"1.0\"}"
  Pipe29_1 : Subsystem  ReferencedSubsystem=PipeSubsystemWithMask  lengthPipe=0.1  areaPipe=3.1416e-06  diaPipe=0.002  directionPipe=up
      settings: PortSchema="{\"entries\":[{\"content\":{\"sides\":[{\"content\":{\"connectorIds\":[\"LConn1\"]},\"type\":\"ConnectorPlacement.EquallySpacedRectSide\",\"uuid\":\"064b9882-c01d-4ca6-b21a-bda87b570164\"},{\"content\":{\"connectorIds\":[\"RConn1\"],\"side\":\"RIGHT\"},\"type\":\"ConnectorPlacement.EquallySpacedRectSide\",\"uuid\":\"eee751c1-0ee2-4a08-90dc-cac4f5822e04\"},{\"content\":{\"connectorIds\":[\"LConn2\"],\"side\":\"TOP\"},\"type\":\"ConnectorPlacement.EquallySpacedRectSide\",\"uuid\":\"508b7d1b-f548-4587-b0be-a567f0211289\"}]},\"type\":\"ConnectorPlacement.EquallySpacedConnector\",\"uuid\":\"7f420bea-eb7e-4a98-ba9c-58ec0a31ea83\"}],\"packageUris\":[\"http://schema.mathworks.com/mf0/Connector/R2020b\"],\"version\":\"1.0\"}"
  Pipe2_1 : Subsystem  ReferencedSubsystem=PipeSubsystemWithMask  lengthPipe=0.35833  areaPipe=3.1416e-06  diaPipe=0.002  directionPipe=right
      settings: PortSchema="{\"entries\":[{\"content\":{\"sides\":[{\"content\":{\"connectorIds\":[\"LConn1\"]},\"type\":\"ConnectorPlacement.EquallySpacedRectSide\",\"uuid\":\"064b9882-c01d-4ca6-b21a-bda87b570164\"},{\"content\":{\"connectorIds\":[\"RConn1\"],\"side\":\"RIGHT\"},\"type\":\"ConnectorPlacement.EquallySpacedRectSide\",\"uuid\":\"eee751c1-0ee2-4a08-90dc-cac4f5822e04\"},{\"content\":{\"connectorIds\":[\"LConn2\"],\"side\":\"TOP\"},\"type\":\"ConnectorPlacement.EquallySpacedRectSide\",\"uuid\":\"508b7d1b-f548-4587-b0be-a567f0211289\"}]},\"type\":\"ConnectorPlacement.EquallySpacedConnector\",\"uuid\":\"7f420bea-eb7e-4a98-ba9c-58ec0a31ea83\"}],\"packageUris\":[\"http://schema.mathworks.com/mf0/Connector/R2020b\"],\"version\":\"1.0\"}"
  Pipe2_{2..5} (4 alike) : Subsystem  ReferencedSubsystem=PipeSubsystemWithMask  lengthPipe=0.38333  areaPipe=3.1416e-06  diaPipe=0.002  directionPipe=right
      settings: PortSchema="{\"entries\":[{\"content\":{\"sides\":[{\"content\":{\"connectorIds\":[\"LConn1\"]},\"type\":\"ConnectorPlacement.EquallySpacedRectSide\",\"uuid\":\"064b9882-c01d-4ca6-b21a-bda87b570164\"},{\"content\":{\"connectorIds\":[\"RConn1\"],\"side\":\"RIGHT\"},\"type\":\"ConnectorPlacement.EquallySpacedRectSide\",\"uuid\":\"eee751c1-0ee2-4a08-90dc-cac4f5822e04\"},{\"content\":{\"connectorIds\":[\"LConn2\"],\"side\":\"TOP\"},\"type\":\"ConnectorPlacement.EquallySpacedRectSide\",\"uuid\":\"508b7d1b-f548-4587-b0be-a567f0211289\"}]},\"type\":\"ConnectorPlacement.EquallySpacedConnector\",\"uuid\":\"7f420bea-eb7e-4a98-ba9c-58ec0a31ea83\"}],\"packageUris\":[\"http://schema.mathworks.com/mf0/Connector/R2020b\"],\"version\":\"1.0\"}"
  Pipe2_6 : Subsystem  ReferencedSubsystem=PipeSubsystemWithMask  lengthPipe=0.35833  areaPipe=3.1416e-06  diaPipe=0.002  directionPipe=right
      settings: PortSchema="{\"entries\":[{\"content\":{\"sides\":[{\"content\":{\"connectorIds\":[\"LConn1\"]},\"type\":\"ConnectorPlacement.EquallySpacedRectSide\",\"uuid\":\"064b9882-c01d-4ca6-b21a-bda87b570164\"},{\"content\":{\"connectorIds\":[\"RConn1\"],\"side\":\"RIGHT\"},\"type\":\"ConnectorPlacement.EquallySpacedRectSide\",\"uuid\":\"eee751c1-0ee2-4a08-90dc-cac4f5822e04\"},{\"content\":{\"connectorIds\":[\"LConn2\"],\"side\":\"TOP\"},\"type\":\"ConnectorPlacement.EquallySpacedRectSide\",\"uuid\":\"508b7d1b-f548-4587-b0be-a567f0211289\"}]},\"type\":\"ConnectorPlacement.EquallySpacedConnector\",\"uuid\":\"7f420bea-eb7e-4a98-ba9c-58ec0a31ea83\"}],\"packageUris\":[\"http://schema.mathworks.com/mf0/Connector/R2020b\"],\"version\":\"1.0\"}"
  Pipe30_1 : Subsystem  ReferencedSubsystem=PipeSubsystemWithMask  lengthPipe=0.04375  areaPipe=3.1416e-06  diaPipe=0.002  directionPipe=up
      settings: PortSchema="{\"entries\":[{\"content\":{\"sides\":[{\"content\":{\"connectorIds\":[\"LConn1\"]},\"type\":\"ConnectorPlacement.EquallySpacedRectSide\",\"uuid\":\"064b9882-c01d-4ca6-b21a-bda87b570164\"},{\"content\":{\"connectorIds\":[\"RConn1\"],\"side\":\"RIGHT\"},\"type\":\"ConnectorPlacement.EquallySpacedRectSide\",\"uuid\":\"eee751c1-0ee2-4a08-90dc-cac4f5822e04\"},{\"content\":{\"connectorIds\":[\"LConn2\"],\"side\":\"TOP\"},\"type\":\"ConnectorPlacement.EquallySpacedRectSide\",\"uuid\":\"508b7d1b-f548-4587-b0be-a567f0211289\"}]},\"type\":\"ConnectorPlacement.EquallySpacedConnector\",\"uuid\":\"7f420bea-eb7e-4a98-ba9c-58ec0a31ea83\"}],\"packageUris\":[\"http://schema.mathworks.com/mf0/Connector/R2020b\"],\"version\":\"1.0\"}"
  Pipe30_2 : Subsystem  ReferencedSubsystem=PipeSubsystemWithMask  lengthPipe=0.05625  areaPipe=3.1416e-06  diaPipe=0.002  directionPipe=up
      settings: PortSchema="{\"entries\":[{\"content\":{\"sides\":[{\"content\":{\"connectorIds\":[\"LConn1\"]},\"type\":\"ConnectorPlacement.EquallySpacedRectSide\",\"uuid\":\"064b9882-c01d-4ca6-b21a-bda87b570164\"},{\"content\":{\"connectorIds\":[\"RConn1\"],\"side\":\"RIGHT\"},\"type\":\"ConnectorPlacement.EquallySpacedRectSide\",\"uuid\":\"eee751c1-0ee2-4a08-90dc-cac4f5822e04\"},{\"content\":{\"connectorIds\":[\"LConn2\"],\"side\":\"TOP\"},\"type\":\"ConnectorPlacement.EquallySpacedRectSide\",\"uuid\":\"508b7d1b-f548-4587-b0be-a567f0211289\"}]},\"type\":\"ConnectorPlacement.EquallySpacedConnector\",\"uuid\":\"7f420bea-eb7e-4a98-ba9c-58ec0a31ea83\"}],\"packageUris\":[\"http://schema.mathworks.com/mf0/Connector/R2020b\"],\"version\":\"1.0\"}"
  Pipe31_1 : Subsystem  ReferencedSubsystem=PipeSubsystemWithMask  lengthPipe=0.1  areaPipe=3.1416e-06  diaPipe=0.002  directionPipe=up
      settings: PortSchema="{\"entries\":[{\"content\":{\"sides\":[{\"content\":{\"connectorIds\":[\"LConn1\"]},\"type\":\"ConnectorPlacement.EquallySpacedRectSide\",\"uuid\":\"064b9882-c01d-4ca6-b21a-bda87b570164\"},{\"content\":{\"connectorIds\":[\"RConn1\"],\"side\":\"RIGHT\"},\"type\":\"ConnectorPlacement.EquallySpacedRectSide\",\"uuid\":\"eee751c1-0ee2-4a08-90dc-cac4f5822e04\"},{\"content\":{\"connectorIds\":[\"LConn2\"],\"side\":\"TOP\"},\"type\":\"ConnectorPlacement.EquallySpacedRectSide\",\"uuid\":\"508b7d1b-f548-4587-b0be-a567f0211289\"}]},\"type\":\"ConnectorPlacement.EquallySpacedConnector\",\"uuid\":\"7f420bea-eb7e-4a98-ba9c-58ec0a31ea83\"}],\"packageUris\":[\"http://schema.mathworks.com/mf0/Connector/R2020b\"],\"version\":\"1.0\"}"
  Pipe32_1 : Subsystem  ReferencedSubsystem=PipeSubsystemWithMask  lengthPipe=0.1  areaPipe=3.1416e-06  diaPipe=0.002  directionPipe=up
      settings: PortSchema="{\"entries\":[{\"content\":{\"sides\":[{\"content\":{\"connectorIds\":[\"LConn1\"]},\"type\":\"ConnectorPlacement.EquallySpacedRectSide\",\"uuid\":\"064b9882-c01d-4ca6-b21a-bda87b570164\"},{\"content\":{\"connectorIds\":[\"RConn1\"],\"side\":\"RIGHT\"},\"type\":\"ConnectorPlacement.EquallySpacedRectSide\",\"uuid\":\"eee751c1-0ee2-4a08-90dc-cac4f5822e04\"},{\"content\":{\"connectorIds\":[\"LConn2\"],\"side\":\"TOP\"},\"type\":\"ConnectorPlacement.EquallySpacedRectSide\",\"uuid\":\"508b7d1b-f548-4587-b0be-a567f0211289\"}]},\"type\":\"ConnectorPlacement.EquallySpacedConnector\",\"uuid\":\"7f420bea-eb7e-4a98-ba9c-58ec0a31ea83\"}],\"packageUris\":[\"http://schema.mathworks.com/mf0/Connector/R2020b\"],\"version\":\"1.0\"}"
  Pipe33_1 : Subsystem  ReferencedSubsystem=PipeSubsystemWithMask  lengthPipe=0.05625  areaPipe=3.1416e-06  diaPipe=0.002  directionPipe=up
      settings: PortSchema="{\"entries\":[{\"content\":{\"sides\":[{\"content\":{\"connectorIds\":[\"LConn1\"]},\"type\":\"ConnectorPlacement.EquallySpacedRectSide\",\"uuid\":\"064b9882-c01d-4ca6-b21a-bda87b570164\"},{\"content\":{\"connectorIds\":[\"RConn1\"],\"side\":\"RIGHT\"},\"type\":\"ConnectorPlacement.EquallySpacedRectSide\",\"uuid\":\"eee751c1-0ee2-4a08-90dc-cac4f5822e04\"},{\"content\":{\"connectorIds\":[\"LConn2\"],\"side\":\"TOP\"},\"type\":\"ConnectorPlacement.EquallySpacedRectSide\",\"uuid\":\"508b7d1b-f548-4587-b0be-a567f0211289\"}]},\"type\":\"ConnectorPlacement.EquallySpacedConnector\",\"uuid\":\"7f420bea-eb7e-4a98-ba9c-58ec0a31ea83\"}],\"packageUris\":[\"http://schema.mathworks.com/mf0/Connector/R2020b\"],\"version\":\"1.0\"}"
  Pipe33_2 : Subsystem  ReferencedSubsystem=PipeSubsystemWithMask  lengthPipe=0.04375  areaPipe=3.1416e-06  diaPipe=0.002  directionPipe=up
      settings: PortSchema="{\"entries\":[{\"content\":{\"sides\":[{\"content\":{\"connectorIds\":[\"LConn1\"]},\"type\":\"ConnectorPlacement.EquallySpacedRectSide\",\"uuid\":\"064b9882-c01d-4ca6-b21a-bda87b570164\"},{\"content\":{\"connectorIds\":[\"RConn1\"],\"side\":\"RIGHT\"},\"type\":\"ConnectorPlacement.EquallySpacedRectSide\",\"uuid\":\"eee751c1-0ee2-4a08-90dc-cac4f5822e04\"},{\"content\":{\"connectorIds\":[\"LConn2\"],\"side\":\"TOP\"},\"type\":\"ConnectorPlacement.EquallySpacedRectSide\",\"uuid\":\"508b7d1b-f548-4587-b0be-a567f0211289\"}]},\"type\":\"ConnectorPlacement.EquallySpacedConnector\",\"uuid\":\"7f420bea-eb7e-4a98-ba9c-58ec0a31ea83\"}],\"packageUris\":[\"http://schema.mathworks.com/mf0/Connector/R2020b\"],\"version\":\"1.0\"}"
  Pipe34_1 : Subsystem  ReferencedSubsystem=PipeSubsystemWithMask  lengthPipe=0.1  areaPipe=3.1416e-06  diaPipe=0.002  directionPipe=up
      settings: PortSchema="{\"entries\":[{\"content\":{\"sides\":[{\"content\":{\"connectorIds\":[\"LConn1\"]},\"type\":\"ConnectorPlacement.EquallySpacedRectSide\",\"uuid\":\"064b9882-c01d-4ca6-b21a-bda87b570164\"},{\"content\":{\"connectorIds\":[\"RConn1\"],\"side\":\"RIGHT\"},\"type\":\"ConnectorPlacement.EquallySpacedRectSide\",\"uuid\":\"eee751c1-0ee2-4a08-90dc-cac4f5822e04\"},{\"content\":{\"connectorIds\":[\"LConn2\"],\"side\":\"TOP\"},\"type\":\"ConnectorPlacement.EquallySpacedRectSide\",\"uuid\":\"508b7d1b-f548-4587-b0be-a567f0211289\"}]},\"type\":\"ConnectorPlacement.EquallySpacedConnector\",\"uuid\":\"7f420bea-eb7e-4a98-ba9c-58ec0a31ea83\"}],\"packageUris\":[\"http://schema.mathworks.com/mf0/Connector/R2020b\"],\"version\":\"1.0\"}"
  Pipe35_1 : Subsystem  ReferencedSubsystem=PipeSubsystemWithMask  lengthPipe=0.0125  areaPipe=3.1416e-06  diaPipe=0.002  directionPipe=up
      settings: PortSchema="{\"entries\":[{\"content\":{\"sides\":[{\"content\":{\"connectorIds\":[\"LConn1\"]},\"type\":\"ConnectorPlacement.EquallySpacedRectSide\",\"uuid\":\"064b9882-c01d-4ca6-b21a-bda87b570164\"},{\"content\":{\"connectorIds\":[\"RConn1\"],\"side\":\"RIGHT\"},\"type\":\"ConnectorPlacement.EquallySpacedRectSide\",\"uuid\":\"eee751c1-0ee2-4a08-90dc-cac4f5822e04\"},{\"content\":{\"connectorIds\":[\"LConn2\"],\"side\":\"TOP\"},\"type\":\"ConnectorPlacement.EquallySpacedRectSide\",\"uuid\":\"508b7d1b-f548-4587-b0be-a567f0211289\"}]},\"type\":\"ConnectorPlacement.EquallySpacedConnector\",\"uuid\":\"7f420bea-eb7e-4a98-ba9c-58ec0a31ea83\"}],\"packageUris\":[\"http://schema.mathworks.com/mf0/Connector/R2020b\"],\"version\":\"1.0\"}"
  Pipe35_2 : Subsystem  ReferencedSubsystem=PipeSubsystemWithMask  lengthPipe=0.0875  areaPipe=3.1416e-06  diaPipe=0.002  directionPipe=up
      settings: PortSchema="{\"entries\":[{\"content\":{\"sides\":[{\"content\":{\"connectorIds\":[\"LConn1\"]},\"type\":\"ConnectorPlacement.EquallySpacedRectSide\",\"uuid\":\"064b9882-c01d-4ca6-b21a-bda87b570164\"},{\"content\":{\"connectorIds\":[\"RConn1\"],\"side\":\"RIGHT\"},\"type\":\"ConnectorPlacement.EquallySpacedRectSide\",\"uuid\":\"eee751c1-0ee2-4a08-90dc-cac4f5822e04\"},{\"content\":{\"connectorIds\":[\"LConn2\"],\"side\":\"TOP\"},\"type\":\"ConnectorPlacement.EquallySpacedRectSide\",\"uuid\":\"508b7d1b-f548-4587-b0be-a567f0211289\"}]},\"type\":\"ConnectorPlacement.EquallySpacedConnector\",\"uuid\":\"7f420bea-eb7e-4a98-ba9c-58ec0a31ea83\"}],\"packageUris\":[\"http://schema.mathworks.com/mf0/Connector/R2020b\"],\"version\":\"1.0\"}"
  Pipe36_1 : Subsystem  ReferencedSubsystem=PipeSubsystemWithMask  lengthPipe=0.06875  areaPipe=3.1416e-06  diaPipe=0.002  directionPipe=up
      settings: PortSchema="{\"entries\":[{\"content\":{\"sides\":[{\"content\":{\"connectorIds\":[\"LConn1\"]},\"type\":\"ConnectorPlacement.EquallySpacedRectSide\",\"uuid\":\"064b9882-c01d-4ca6-b21a-bda87b570164\"},{\"content\":{\"connectorIds\":[\"RConn1\"],\"side\":\"RIGHT\"},\"type\":\"ConnectorPlacement.EquallySpacedRectSide\",\"uuid\":\"eee751c1-0ee2-4a08-90dc-cac4f5822e04\"},{\"content\":{\"connectorIds\":[\"LConn2\"],\"side\":\"TOP\"},\"type\":\"ConnectorPlacement.EquallySpacedRectSide\",\"uuid\":\"508b7d1b-f548-4587-b0be-a567f0211289\"}]},\"type\":\"ConnectorPlacement.EquallySpacedConnector\",\"uuid\":\"7f420bea-eb7e-4a98-ba9c-58ec0a31ea83\"}],\"packageUris\":[\"http://schema.mathworks.com/mf0/Connector/R2020b\"],\"version\":\"1.0\"}"
  Pipe36_2 : Subsystem  ReferencedSubsystem=PipeSubsystemWithMask  lengthPipe=0.03125  areaPipe=3.1416e-06  diaPipe=0.002  directionPipe=up
      settings: PortSchema="{\"entries\":[{\"content\":{\"sides\":[{\"content\":{\"connectorIds\":[\"LConn1\"]},\"type\":\"ConnectorPlacement.EquallySpacedRectSide\",\"uuid\":\"064b9882-c01d-4ca6-b21a-bda87b570164\"},{\"content\":{\"connectorIds\":[\"RConn1\"],\"side\":\"RIGHT\"},\"type\":\"ConnectorPlacement.EquallySpacedRectSide\",\"uuid\":\"eee751c1-0ee2-4a08-90dc-cac4f5822e04\"},{\"content\":{\"connectorIds\":[\"LConn2\"],\"side\":\"TOP\"},\"type\":\"ConnectorPlacement.EquallySpacedRectSide\",\"uuid\":\"508b7d1b-f548-4587-b0be-a567f0211289\"}]},\"type\":\"ConnectorPlacement.EquallySpacedConnector\",\"uuid\":\"7f420bea-eb7e-4a98-ba9c-58ec0a31ea83\"}],\"packageUris\":[\"http://schema.mathworks.com/mf0/Connector/R2020b\"],\"version\":\"1.0\"}"
  Pipe37_1 : Subsystem  ReferencedSubsystem=PipeSubsystemWithMask  lengthPipe=0.1  areaPipe=3.1416e-06  diaPipe=0.002  directionPipe=up
      settings: PortSchema="{\"entries\":[{\"content\":{\"sides\":[{\"content\":{\"connectorIds\":[\"LConn1\"]},\"type\":\"ConnectorPlacement.EquallySpacedRectSide\",\"uuid\":\"064b9882-c01d-4ca6-b21a-bda87b570164\"},{\"content\":{\"connectorIds\":[\"RConn1\"],\"side\":\"RIGHT\"},\"type\":\"ConnectorPlacement.EquallySpacedRectSide\",\"uuid\":\"eee751c1-0ee2-4a08-90dc-cac4f5822e04\"},{\"content\":{\"connectorIds\":[\"LConn2\"],\"side\":\"TOP\"},\"type\":\"ConnectorPlacement.EquallySpacedRectSide\",\"uuid\":\"508b7d1b-f548-4587-b0be-a567f0211289\"}]},\"type\":\"ConnectorPlacement.EquallySpacedConnector\",\"uuid\":\"7f420bea-eb7e-4a98-ba9c-58ec0a31ea83\"}],\"packageUris\":[\"http://schema.mathworks.com/mf0/Connector/R2020b\"],\"version\":\"1.0\"}"
  Pipe3_1 : Subsystem  ReferencedSubsystem=PipeSubsystemWithMask  lengthPipe=0.35833  areaPipe=3.1416e-06  diaPipe=0.002  directionPipe=right
      settings: PortSchema="{\"entries\":[{\"content\":{\"sides\":[{\"content\":{\"connectorIds\":[\"LConn1\"]},\"type\":\"ConnectorPlacement.EquallySpacedRectSide\",\"uuid\":\"064b9882-c01d-4ca6-b21a-bda87b570164\"},{\"content\":{\"connectorIds\":[\"RConn1\"],\"side\":\"RIGHT\"},\"type\":\"ConnectorPlacement.EquallySpacedRectSide\",\"uuid\":\"eee751c1-0ee2-4a08-90dc-cac4f5822e04\"},{\"content\":{\"connectorIds\":[\"LConn2\"],\"side\":\"TOP\"},\"type\":\"ConnectorPlacement.EquallySpacedRectSide\",\"uuid\":\"508b7d1b-f548-4587-b0be-a567f0211289\"}]},\"type\":\"ConnectorPlacement.EquallySpacedConnector\",\"uuid\":\"7f420bea-eb7e-4a98-ba9c-58ec0a31ea83\"}],\"packageUris\":[\"http://schema.mathworks.com/mf0/Connector/R2020b\"],\"version\":\"1.0\"}"
  Pipe3_{2..5} (4 alike) : Subsystem  ReferencedSubsystem=PipeSubsystemWithMask  lengthPipe=0.38333  areaPipe=3.1416e-06  diaPipe=0.002  directionPipe=right
      settings: PortSchema="{\"entries\":[{\"content\":{\"sides\":[{\"content\":{\"connectorIds\":[\"LConn1\"]},\"type\":\"ConnectorPlacement.EquallySpacedRectSide\",\"uuid\":\"064b9882-c01d-4ca6-b21a-bda87b570164\"},{\"content\":{\"connectorIds\":[\"RConn1\"],\"side\":\"RIGHT\"},\"type\":\"ConnectorPlacement.EquallySpacedRectSide\",\"uuid\":\"eee751c1-0ee2-4a08-90dc-cac4f5822e04\"},{\"content\":{\"connectorIds\":[\"LConn2\"],\"side\":\"TOP\"},\"type\":\"ConnectorPlacement.EquallySpacedRectSide\",\"uuid\":\"508b7d1b-f548-4587-b0be-a567f0211289\"}]},\"type\":\"ConnectorPlacement.EquallySpacedConnector\",\"uuid\":\"7f420bea-eb7e-4a98-ba9c-58ec0a31ea83\"}],\"packageUris\":[\"http://schema.mathworks.com/mf0/Connector/R2020b\"],\"version\":\"1.0\"}"
  Pipe3_6 : Subsystem  ReferencedSubsystem=PipeSubsystemWithMask  lengthPipe=0.35833  areaPipe=3.1416e-06  diaPipe=0.002  directionPipe=right
      settings: PortSchema="{\"entries\":[{\"content\":{\"sides\":[{\"content\":{\"connectorIds\":[\"LConn1\"]},\"type\":\"ConnectorPlacement.EquallySpacedRectSide\",\"uuid\":\"064b9882-c01d-4ca6-b21a-bda87b570164\"},{\"content\":{\"connectorIds\":[\"RConn1\"],\"side\":\"RIGHT\"},\"type\":\"ConnectorPlacement.EquallySpacedRectSide\",\"uuid\":\"eee751c1-0ee2-4a08-90dc-cac4f5822e04\"},{\"content\":{\"connectorIds\":[\"LConn2\"],\"side\":\"TOP\"},\"type\":\"ConnectorPlacement.EquallySpacedRectSide\",\"uuid\":\"508b7d1b-f548-4587-b0be-a567f0211289\"}]},\"type\":\"ConnectorPlacement.EquallySpacedConnector\",\"uuid\":\"7f420bea-eb7e-4a98-ba9c-58ec0a31ea83\"}],\"packageUris\":[\"http://schema.mathworks.com/mf0/Connector/R2020b\"],\"version\":\"1.0\"}"
  Pipe4_1 : Subsystem  ReferencedSubsystem=PipeSubsystemWithMask  lengthPipe=0.35833  areaPipe=3.1416e-06  diaPipe=0.002  directionPipe=right
      settings: PortSchema="{\"entries\":[{\"content\":{\"sides\":[{\"content\":{\"connectorIds\":[\"LConn1\"]},\"type\":\"ConnectorPlacement.EquallySpacedRectSide\",\"uuid\":\"064b9882-c01d-4ca6-b21a-bda87b570164\"},{\"content\":{\"connectorIds\":[\"RConn1\"],\"side\":\"RIGHT\"},\"type\":\"ConnectorPlacement.EquallySpacedRectSide\",\"uuid\":\"eee751c1-0ee2-4a08-90dc-cac4f5822e04\"},{\"content\":{\"connectorIds\":[\"LConn2\"],\"side\":\"TOP\"},\"type\":\"ConnectorPlacement.EquallySpacedRectSide\",\"uuid\":\"508b7d1b-f548-4587-b0be-a567f0211289\"}]},\"type\":\"ConnectorPlacement.EquallySpacedConnector\",\"uuid\":\"7f420bea-eb7e-4a98-ba9c-58ec0a31ea83\"}],\"packageUris\":[\"http://schema.mathworks.com/mf0/Connector/R2020b\"],\"version\":\"1.0\"}"
  Pipe4_{2..5} (4 alike) : Subsystem  ReferencedSubsystem=PipeSubsystemWithMask  lengthPipe=0.38333  areaPipe=3.1416e-06  diaPipe=0.002  directionPipe=right
      settings: PortSchema="{\"entries\":[{\"content\":{\"sides\":[{\"content\":{\"connectorIds\":[\"LConn1\"]},\"type\":\"ConnectorPlacement.EquallySpacedRectSide\",\"uuid\":\"064b9882-c01d-4ca6-b21a-bda87b570164\"},{\"content\":{\"connectorIds\":[\"RConn1\"],\"side\":\"RIGHT\"},\"type\":\"ConnectorPlacement.EquallySpacedRectSide\",\"uuid\":\"eee751c1-0ee2-4a08-90dc-cac4f5822e04\"},{\"content\":{\"connectorIds\":[\"LConn2\"],\"side\":\"TOP\"},\"type\":\"ConnectorPlacement.EquallySpacedRectSide\",\"uuid\":\"508b7d1b-f548-4587-b0be-a567f0211289\"}]},\"type\":\"ConnectorPlacement.EquallySpacedConnector\",\"uuid\":\"7f420bea-eb7e-4a98-ba9c-58ec0a31ea83\"}],\"packageUris\":[\"http://schema.mathworks.com/mf0/Connector/R2020b\"],\"version\":\"1.0\"}"
  Pipe4_6 : Subsystem  ReferencedSubsystem=PipeSubsystemWithMask  lengthPipe=0.35833  areaPipe=3.1416e-06  diaPipe=0.002  directionPipe=right
      settings: PortSchema="{\"entries\":[{\"content\":{\"sides\":[{\"content\":{\"connectorIds\":[\"LConn1\"]},\"type\":\"ConnectorPlacement.EquallySpacedRectSide\",\"uuid\":\"064b9882-c01d-4ca6-b21a-bda87b570164\"},{\"content\":{\"connectorIds\":[\"RConn1\"],\"side\":\"RIGHT\"},\"type\":\"ConnectorPlacement.EquallySpacedRectSide\",\"uuid\":\"eee751c1-0ee2-4a08-90dc-cac4f5822e04\"},{\"content\":{\"connectorIds\":[\"LConn2\"],\"side\":\"TOP\"},\"type\":\"ConnectorPlacement.EquallySpacedRectSide\",\"uuid\":\"508b7d1b-f548-4587-b0be-a567f0211289\"}]},\"type\":\"ConnectorPlacement.EquallySpacedConnector\",\"uuid\":\"7f420bea-eb7e-4a98-ba9c-58ec0a31ea83\"}],\"packageUris\":[\"http://schema.mathworks.com/mf0/Connector/R2020b\"],\"version\":\"1.0\"}"
  Pipe5_1 : Subsystem  ReferencedSubsystem=PipeSubsystemWithMask  lengthPipe=0.35833  areaPipe=3.1416e-06  diaPipe=0.002  directionPipe=right
      settings: PortSchema="{\"entries\":[{\"content\":{\"sides\":[{\"content\":{\"connectorIds\":[\"LConn1\"]},\"type\":\"ConnectorPlacement.EquallySpacedRectSide\",\"uuid\":\"064b9882-c01d-4ca6-b21a-bda87b570164\"},{\"content\":{\"connectorIds\":[\"RConn1\"],\"side\":\"RIGHT\"},\"type\":\"ConnectorPlacement.EquallySpacedRectSide\",\"uuid\":\"eee751c1-0ee2-4a08-90dc-cac4f5822e04\"},{\"content\":{\"connectorIds\":[\"LConn2\"],\"side\":\"TOP\"},\"type\":\"ConnectorPlacement.EquallySpacedRectSide\",\"uuid\":\"508b7d1b-f548-4587-b0be-a567f0211289\"}]},\"type\":\"ConnectorPlacement.EquallySpacedConnector\",\"uuid\":\"7f420bea-eb7e-4a98-ba9c-58ec0a31ea83\"}],\"packageUris\":[\"http://schema.mathworks.com/mf0/Connector/R2020b\"],\"version\":\"1.0\"}"
  Pipe5_{2..5} (4 alike) : Subsystem  ReferencedSubsystem=PipeSubsystemWithMask  lengthPipe=0.38333  areaPipe=3.1416e-06  diaPipe=0.002  directionPipe=right
      settings: PortSchema="{\"entries\":[{\"content\":{\"sides\":[{\"content\":{\"connectorIds\":[\"LConn1\"]},\"type\":\"ConnectorPlacement.EquallySpacedRectSide\",\"uuid\":\"064b9882-c01d-4ca6-b21a-bda87b570164\"},{\"content\":{\"connectorIds\":[\"RConn1\"],\"side\":\"RIGHT\"},\"type\":\"ConnectorPlacement.EquallySpacedRectSide\",\"uuid\":\"eee751c1-0ee2-4a08-90dc-cac4f5822e04\"},{\"content\":{\"connectorIds\":[\"LConn2\"],\"side\":\"TOP\"},\"type\":\"ConnectorPlacement.EquallySpacedRectSide\",\"uuid\":\"508b7d1b-f548-4587-b0be-a567f0211289\"}]},\"type\":\"ConnectorPlacement.EquallySpacedConnector\",\"uuid\":\"7f420bea-eb7e-4a98-ba9c-58ec0a31ea83\"}],\"packageUris\":[\"http://schema.mathworks.com/mf0/Connector/R2020b\"],\"version\":\"1.0\"}"
  Pipe5_6 : Subsystem  ReferencedSubsystem=PipeSubsystemWithMask  lengthPipe=0.35833  areaPipe=3.1416e-06  diaPipe=0.002  directionPipe=right
      settings: PortSchema="{\"entries\":[{\"content\":{\"sides\":[{\"content\":{\"connectorIds\":[\"LConn1\"]},\"type\":\"ConnectorPlacement.EquallySpacedRectSide\",\"uuid\":\"064b9882-c01d-4ca6-b21a-bda87b570164\"},{\"content\":{\"connectorIds\":[\"RConn1\"],\"side\":\"RIGHT\"},\"type\":\"ConnectorPlacement.EquallySpacedRectSide\",\"uuid\":\"eee751c1-0ee2-4a08-90dc-cac4f5822e04\"},{\"content\":{\"connectorIds\":[\"LConn2\"],\"side\":\"TOP\"},\"type\":\"ConnectorPlacement.EquallySpacedRectSide\",\"uuid\":\"508b7d1b-f548-4587-b0be-a567f0211289\"}]},\"type\":\"ConnectorPlacement.EquallySpacedConnector\",\"uuid\":\"7f420bea-eb7e-4a98-ba9c-58ec0a31ea83\"}],\"packageUris\":[\"http://schema.mathworks.com/mf0/Connector/R2020b\"],\"version\":\"1.0\"}"
  Pipe6_1 : Subsystem  ReferencedSubsystem=PipeSubsystemWithMask  lengthPipe=0.35833  areaPipe=3.1416e-06  diaPipe=0.002  directionPipe=right
      settings: PortSchema="{\"entries\":[{\"content\":{\"sides\":[{\"content\":{\"connectorIds\":[\"LConn1\"]},\"type\":\"ConnectorPlacement.EquallySpacedRectSide\",\"uuid\":\"064b9882-c01d-4ca6-b21a-bda87b570164\"},{\"content\":{\"connectorIds\":[\"RConn1\"],\"side\":\"RIGHT\"},\"type\":\"ConnectorPlacement.EquallySpacedRectSide\",\"uuid\":\"eee751c1-0ee2-4a08-90dc-cac4f5822e04\"},{\"content\":{\"connectorIds\":[\"LConn2\"],\"side\":\"TOP\"},\"type\":\"ConnectorPlacement.EquallySpacedRectSide\",\"uuid\":\"508b7d1b-f548-4587-b0be-a567f0211289\"}]},\"type\":\"ConnectorPlacement.EquallySpacedConnector\",\"uuid\":\"7f420bea-eb7e-4a98-ba9c-58ec0a31ea83\"}],\"packageUris\":[\"http://schema.mathworks.com/mf0/Connector/R2020b\"],\"version\":\"1.0\"}"
  Pipe6_{2..5} (4 alike) : Subsystem  ReferencedSubsystem=PipeSubsystemWithMask  lengthPipe=0.38333  areaPipe=3.1416e-06  diaPipe=0.002  directionPipe=right
      settings: PortSchema="{\"entries\":[{\"content\":{\"sides\":[{\"content\":{\"connectorIds\":[\"LConn1\"]},\"type\":\"ConnectorPlacement.EquallySpacedRectSide\",\"uuid\":\"064b9882-c01d-4ca6-b21a-bda87b570164\"},{\"content\":{\"connectorIds\":[\"RConn1\"],\"side\":\"RIGHT\"},\"type\":\"ConnectorPlacement.EquallySpacedRectSide\",\"uuid\":\"eee751c1-0ee2-4a08-90dc-cac4f5822e04\"},{\"content\":{\"connectorIds\":[\"LConn2\"],\"side\":\"TOP\"},\"type\":\"ConnectorPlacement.EquallySpacedRectSide\",\"uuid\":\"508b7d1b-f548-4587-b0be-a567f0211289\"}]},\"type\":\"ConnectorPlacement.EquallySpacedConnector\",\"uuid\":\"7f420bea-eb7e-4a98-ba9c-58ec0a31ea83\"}],\"packageUris\":[\"http://schema.mathworks.com/mf0/Connector/R2020b\"],\"version\":\"1.0\"}"
  Pipe6_6 : Subsystem  ReferencedSubsystem=PipeSubsystemWithMask  lengthPipe=0.35833  areaPipe=3.1416e-06  diaPipe=0.002  directionPipe=right
      settings: PortSchema="{\"entries\":[{\"content\":{\"sides\":[{\"content\":{\"connectorIds\":[\"LConn1\"]},\"type\":\"ConnectorPlacement.EquallySpacedRectSide\",\"uuid\":\"064b9882-c01d-4ca6-b21a-bda87b570164\"},{\"content\":{\"connectorIds\":[\"RConn1\"],\"side\":\"RIGHT\"},\"type\":\"ConnectorPlacement.EquallySpacedRectSide\",\"uuid\":\"eee751c1-0ee2-4a08-90dc-cac4f5822e04\"},{\"content\":{\"connectorIds\":[\"LConn2\"],\"side\":\"TOP\"},\"type\":\"ConnectorPlacement.EquallySpacedRectSide\",\"uuid\":\"508b7d1b-f548-4587-b0be-a567f0211289\"}]},\"type\":\"ConnectorPlacement.EquallySpacedConnector\",\"uuid\":\"7f420bea-eb7e-4a98-ba9c-58ec0a31ea83\"}],\"packageUris\":[\"http://schema.mathworks.com/mf0/Connector/R2020b\"],\"version\":\"1.0\"}"
  Pipe7_1 : Subsystem  ReferencedSubsystem=PipeSubsystemWithMask  lengthPipe=0.35833  areaPipe=3.1416e-06  diaPipe=0.002  directionPipe=right
      settings: PortSchema="{\"entries\":[{\"content\":{\"sides\":[{\"content\":{\"connectorIds\":[\"LConn1\"]},\"type\":\"ConnectorPlacement.EquallySpacedRectSide\",\"uuid\":\"064b9882-c01d-4ca6-b21a-bda87b570164\"},{\"content\":{\"connectorIds\":[\"RConn1\"],\"side\":\"RIGHT\"},\"type\":\"ConnectorPlacement.EquallySpacedRectSide\",\"uuid\":\"eee751c1-0ee2-4a08-90dc-cac4f5822e04\"},{\"content\":{\"connectorIds\":[\"LConn2\"],\"side\":\"TOP\"},\"type\":\"ConnectorPlacement.EquallySpacedRectSide\",\"uuid\":\"508b7d1b-f548-4587-b0be-a567f0211289\"}]},\"type\":\"ConnectorPlacement.EquallySpacedConnector\",\"uuid\":\"7f420bea-eb7e-4a98-ba9c-58ec0a31ea83\"}],\"packageUris\":[\"http://schema.mathworks.com/mf0/Connector/R2020b\"],\"version\":\"1.0\"}"
  Pipe7_{2..5} (4 alike) : Subsystem  ReferencedSubsystem=PipeSubsystemWithMask  lengthPipe=0.38333  areaPipe=3.1416e-06  diaPipe=0.002  directionPipe=right
      settings: PortSchema="{\"entries\":[{\"content\":{\"sides\":[{\"content\":{\"connectorIds\":[\"LConn1\"]},\"type\":\"ConnectorPlacement.EquallySpacedRectSide\",\"uuid\":\"064b9882-c01d-4ca6-b21a-bda87b570164\"},{\"content\":{\"connectorIds\":[\"RConn1\"],\"side\":\"RIGHT\"},\"type\":\"ConnectorPlacement.EquallySpacedRectSide\",\"uuid\":\"eee751c1-0ee2-4a08-90dc-cac4f5822e04\"},{\"content\":{\"connectorIds\":[\"LConn2\"],\"side\":\"TOP\"},\"type\":\"ConnectorPlacement.EquallySpacedRectSide\",\"uuid\":\"508b7d1b-f548-4587-b0be-a567f0211289\"}]},\"type\":\"ConnectorPlacement.EquallySpacedConnector\",\"uuid\":\"7f420bea-eb7e-4a98-ba9c-58ec0a31ea83\"}],\"packageUris\":[\"http://schema.mathworks.com/mf0/Connector/R2020b\"],\"version\":\"1.0\"}"
  Pipe7_6 : Subsystem  ReferencedSubsystem=PipeSubsystemWithMask  lengthPipe=0.35833  areaPipe=3.1416e-06  diaPipe=0.002  directionPipe=right
      settings: PortSchema="{\"entries\":[{\"content\":{\"sides\":[{\"content\":{\"connectorIds\":[\"LConn1\"]},\"type\":\"ConnectorPlacement.EquallySpacedRectSide\",\"uuid\":\"064b9882-c01d-4ca6-b21a-bda87b570164\"},{\"content\":{\"connectorIds\":[\"RConn1\"],\"side\":\"RIGHT\"},\"type\":\"ConnectorPlacement.EquallySpacedRectSide\",\"uuid\":\"eee751c1-0ee2-4a08-90dc-cac4f5822e04\"},{\"content\":{\"connectorIds\":[\"LConn2\"],\"side\":\"TOP\"},\"type\":\"ConnectorPlacement.EquallySpacedRectSide\",\"uuid\":\"508b7d1b-f548-4587-b0be-a567f0211289\"}]},\"type\":\"ConnectorPlacement.EquallySpacedConnector\",\"uuid\":\"7f420bea-eb7e-4a98-ba9c-58ec0a31ea83\"}],\"packageUris\":[\"http://schema.mathworks.com/mf0/Connector/R2020b\"],\"version\":\"1.0\"}"
  Pipe8_1 : Subsystem  ReferencedSubsystem=PipeSubsystemWithMask  lengthPipe=0.35833  areaPipe=3.1416e-06  diaPipe=0.002  directionPipe=right
      settings: PortSchema="{\"entries\":[{\"content\":{\"sides\":[{\"content\":{\"connectorIds\":[\"LConn1\"]},\"type\":\"ConnectorPlacement.EquallySpacedRectSide\",\"uuid\":\"064b9882-c01d-4ca6-b21a-bda87b570164\"},{\"content\":{\"connectorIds\":[\"RConn1\"],\"side\":\"RIGHT\"},\"type\":\"ConnectorPlacement.EquallySpacedRectSide\",\"uuid\":\"eee751c1-0ee2-4a08-90dc-cac4f5822e04\"},{\"content\":{\"connectorIds\":[\"LConn2\"],\"side\":\"TOP\"},\"type\":\"ConnectorPlacement.EquallySpacedRectSide\",\"uuid\":\"508b7d1b-f548-4587-b0be-a567f0211289\"}]},\"type\":\"ConnectorPlacement.EquallySpacedConnector\",\"uuid\":\"7f420bea-eb7e-4a98-ba9c-58ec0a31ea83\"}],\"packageUris\":[\"http://schema.mathworks.com/mf0/Connector/R2020b\"],\"version\":\"1.0\"}"
  Pipe8_{2..5} (4 alike) : Subsystem  ReferencedSubsystem=PipeSubsystemWithMask  lengthPipe=0.38333  areaPipe=3.1416e-06  diaPipe=0.002  directionPipe=right
      settings: PortSchema="{\"entries\":[{\"content\":{\"sides\":[{\"content\":{\"connectorIds\":[\"LConn1\"]},\"type\":\"ConnectorPlacement.EquallySpacedRectSide\",\"uuid\":\"064b9882-c01d-4ca6-b21a-bda87b570164\"},{\"content\":{\"connectorIds\":[\"RConn1\"],\"side\":\"RIGHT\"},\"type\":\"ConnectorPlacement.EquallySpacedRectSide\",\"uuid\":\"eee751c1-0ee2-4a08-90dc-cac4f5822e04\"},{\"content\":{\"connectorIds\":[\"LConn2\"],\"side\":\"TOP\"},\"type\":\"ConnectorPlacement.EquallySpacedRectSide\",\"uuid\":\"508b7d1b-f548-4587-b0be-a567f0211289\"}]},\"type\":\"ConnectorPlacement.EquallySpacedConnector\",\"uuid\":\"7f420bea-eb7e-4a98-ba9c-58ec0a31ea83\"}],\"packageUris\":[\"http://schema.mathworks.com/mf0/Connector/R2020b\"],\"version\":\"1.0\"}"
  Pipe8_6 : Subsystem  ReferencedSubsystem=PipeSubsystemWithMask  lengthPipe=0.35833  areaPipe=3.1416e-06  diaPipe=0.002  directionPipe=right
      settings: PortSchema="{\"entries\":[{\"content\":{\"sides\":[{\"content\":{\"connectorIds\":[\"LConn1\"]},\"type\":\"ConnectorPlacement.EquallySpacedRectSide\",\"uuid\":\"064b9882-c01d-4ca6-b21a-bda87b570164\"},{\"content\":{\"connectorIds\":[\"RConn1\"],\"side\":\"RIGHT\"},\"type\":\"ConnectorPlacement.EquallySpacedRectSide\",\"uuid\":\"eee751c1-0ee2-4a08-90dc-cac4f5822e04\"},{\"content\":{\"connectorIds\":[\"LConn2\"],\"side\":\"TOP\"},\"type\":\"ConnectorPlacement.EquallySpacedRectSide\",\"uuid\":\"508b7d1b-f548-4587-b0be-a567f0211289\"}]},\"type\":\"ConnectorPlacement.EquallySpacedConnector\",\"uuid\":\"7f420bea-eb7e-4a98-ba9c-58ec0a31ea83\"}],\"packageUris\":[\"http://schema.mathworks.com/mf0/Connector/R2020b\"],\"version\":\"1.0\"}"
  Pipe9_1 : Subsystem  ReferencedSubsystem=PipeSubsystemWithMask  lengthPipe=0.35833  areaPipe=3.1416e-06  diaPipe=0.002  directionPipe=right
      settings: PortSchema="{\"entries\":[{\"content\":{\"sides\":[{\"content\":{\"connectorIds\":[\"LConn1\"]},\"type\":\"ConnectorPlacement.EquallySpacedRectSide\",\"uuid\":\"064b9882-c01d-4ca6-b21a-bda87b570164\"},{\"content\":{\"connectorIds\":[\"RConn1\"],\"side\":\"RIGHT\"},\"type\":\"ConnectorPlacement.EquallySpacedRectSide\",\"uuid\":\"eee751c1-0ee2-4a08-90dc-cac4f5822e04\"},{\"content\":{\"connectorIds\":[\"LConn2\"],\"side\":\"TOP\"},\"type\":\"ConnectorPlacement.EquallySpacedRectSide\",\"uuid\":\"508b7d1b-f548-4587-b0be-a567f0211289\"}]},\"type\":\"ConnectorPlacement.EquallySpacedConnector\",\"uuid\":\"7f420bea-eb7e-4a98-ba9c-58ec0a31ea83\"}],\"packageUris\":[\"http://schema.mathworks.com/mf0/Connector/R2020b\"],\"version\":\"1.0\"}"
  Pipe9_{2..5} (4 alike) : Subsystem  ReferencedSubsystem=PipeSubsystemWithMask  lengthPipe=0.38333  areaPipe=3.1416e-06  diaPipe=0.002  directionPipe=right
      settings: PortSchema="{\"entries\":[{\"content\":{\"sides\":[{\"content\":{\"connectorIds\":[\"LConn1\"]},\"type\":\"ConnectorPlacement.EquallySpacedRectSide\",\"uuid\":\"064b9882-c01d-4ca6-b21a-bda87b570164\"},{\"content\":{\"connectorIds\":[\"RConn1\"],\"side\":\"RIGHT\"},\"type\":\"ConnectorPlacement.EquallySpacedRectSide\",\"uuid\":\"eee751c1-0ee2-4a08-90dc-cac4f5822e04\"},{\"content\":{\"connectorIds\":[\"LConn2\"],\"side\":\"TOP\"},\"type\":\"ConnectorPlacement.EquallySpacedRectSide\",\"uuid\":\"508b7d1b-f548-4587-b0be-a567f0211289\"}]},\"type\":\"ConnectorPlacement.EquallySpacedConnector\",\"uuid\":\"7f420bea-eb7e-4a98-ba9c-58ec0a31ea83\"}],\"packageUris\":[\"http://schema.mathworks.com/mf0/Connector/R2020b\"],\"version\":\"1.0\"}"
  Pipe9_6 : Subsystem  ReferencedSubsystem=PipeSubsystemWithMask  lengthPipe=0.35833  areaPipe=3.1416e-06  diaPipe=0.002  directionPipe=right
      settings: PortSchema="{\"entries\":[{\"content\":{\"sides\":[{\"content\":{\"connectorIds\":[\"LConn1\"]},\"type\":\"ConnectorPlacement.EquallySpacedRectSide\",\"uuid\":\"064b9882-c01d-4ca6-b21a-bda87b570164\"},{\"content\":{\"connectorIds\":[\"RConn1\"],\"side\":\"RIGHT\"},\"type\":\"ConnectorPlacement.EquallySpacedRectSide\",\"uuid\":\"eee751c1-0ee2-4a08-90dc-cac4f5822e04\"},{\"content\":{\"connectorIds\":[\"LConn2\"],\"side\":\"TOP\"},\"type\":\"ConnectorPlacement.EquallySpacedRectSide\",\"uuid\":\"508b7d1b-f548-4587-b0be-a567f0211289\"}]},\"type\":\"ConnectorPlacement.EquallySpacedConnector\",\"uuid\":\"7f420bea-eb7e-4a98-ba9c-58ec0a31ea83\"}],\"packageUris\":[\"http://schema.mathworks.com/mf0/Connector/R2020b\"],\"version\":\"1.0\"}"
  fluid_in : PMIOPort  Side=Left
  fluid_out : PMIOPort  Port=2  Side=Right
  H : PMIOPort  Port=3  Side=Left
  connections:
  Array Connection/RConn1 -- H/RConn1
  H_39_1_bus/LConn1 -- Array Connection/LConn116
  Bend2_1/RConn1 -- H_39_1/LConn1
  H_38_1_bus/LConn1 -- Array Connection/LConn115
  Bend1_1/RConn1 -- H_38_1/LConn1
  H_37_1_bus/LConn1 -- Array Connection/LConn114
  Pipe37_1/LConn2 -- H_37_1/LConn1
  H_36_2_bus/LConn1 -- Array Connection/LConn113
  Pipe36_2/LConn2 -- H_36_2/LConn1
  H_36_1_bus/LConn1 -- Array Connection/LConn112
  Pipe36_1/LConn2 -- H_36_1/LConn1
  Pipe36_1/RConn1 -- Pipe36_2/LConn1
  H_35_2_bus/LConn1 -- Array Connection/LConn111
  Pipe35_2/LConn2 -- H_35_2/LConn1
  H_35_1_bus/LConn1 -- Array Connection/LConn110
  Pipe35_1/LConn2 -- H_35_1/LConn1
  Pipe35_1/RConn1 -- Pipe35_2/LConn1
  H_34_1_bus/LConn1 -- Array Connection/LConn109
  Pipe34_1/LConn2 -- H_34_1/LConn1
  H_33_2_bus/LConn1 -- Array Connection/LConn108
  Pipe33_2/LConn2 -- H_33_2/LConn1
  H_33_1_bus/LConn1 -- Array Connection/LConn107
  Pipe33_1/LConn2 -- H_33_1/LConn1
  Pipe33_1/RConn1 -- Pipe33_2/LConn1
  H_32_1_bus/LConn1 -- Array Connection/LConn106
  Pipe32_1/LConn2 -- H_32_1/LConn1
  H_31_1_bus/LConn1 -- Array Connection/LConn105
  Pipe31_1/LConn2 -- H_31_1/LConn1
  H_30_2_bus/LConn1 -- Array Connection/LConn104
  Pipe30_2/LConn2 -- H_30_2/LConn1
  H_30_1_bus/LConn1 -- Array Connection/LConn103
  Pipe30_1/LConn2 -- H_30_1/LConn1
  Pipe30_1/RConn1 -- Pipe30_2/LConn1
  H_29_1_bus/LConn1 -- Array Connection/LConn102
  Pipe29_1/LConn2 -- H_29_1/LConn1
  H_28_2_bus/LConn1 -- Array Connection/LConn101
  Pipe28_2/LConn2 -- H_28_2/LConn1
  H_28_1_bus/LConn1 -- Array Connection/LConn100
  Pipe28_1/LConn2 -- H_28_1/LConn1
  Pipe28_1/RConn1 -- Pipe28_2/LConn1
  H_27_2_bus/LConn1 -- Array Connection/LConn99
  Pipe27_2/LConn2 -- H_27_2/LConn1
  H_27_1_bus/LConn1 -- Array Connection/LConn98
  Pipe27_1/LConn2 -- H_27_1/LConn1
  Pipe27_1/RConn1 -- Pipe27_2/LConn1
  Pipe26_1/LConn1 -- Bend2_1/LConn2
  H_26_1_bus/LConn1 -- Array Connection/LConn97
  Pipe26_1/LConn2 -- H_26_1/LConn1
  Pipe25_1/RConn1 -- Bend1_1/LConn1
  H_25_1_bus/LConn1 -- Array Connection/LConn96
  Pipe25_1/LConn2 -- H_25_1/LConn1
  H_24_2_bus/LConn1 -- Array Connection/LConn95
  Pipe24_2/LConn2 -- H_24_2/LConn1
  H_24_1_bus/LConn1 -- Array Connection/LConn94
  Pipe24_1/LConn2 -- H_24_1/LConn1
  Pipe24_1/RConn1 -- Pipe24_2/LConn1
  H_23_2_bus/LConn1 -- Array Connection/LConn93
  Pipe23_2/LConn2 -- H_23_2/LConn1
  H_23_1_bus/LConn1 -- Array Connection/LConn92
  Pipe23_1/LConn2 -- H_23_1/LConn1
  Pipe23_1/RConn1 -- Pipe23_2/LConn1
  H_22_1_bus/LConn1 -- Array Connection/LConn91
  Pipe22_1/LConn2 -- H_22_1/LConn1
  H_21_2_bus/LConn1 -- Array Connection/LConn90
  Pipe21_2/LConn2 -- H_21_2/LConn1
  H_21_1_bus/LConn1 -- Array Connection/LConn89
  Pipe21_1/LConn2 -- H_21_1/LConn1
  Pipe21_1/RConn1 -- Pipe21_2/LConn1
  H_20_1_bus/LConn1 -- Array Connection/LConn88
  Pipe20_1/LConn2 -- H_20_1/LConn1
  H_19_1_bus/LConn1 -- Array Connection/LConn87
  Pipe19_1/LConn2 -- H_19_1/LConn1
  H_18_2_bus/LConn1 -- Array Connection/LConn86
  Pipe18_2/LConn2 -- H_18_2/LConn1
  H_18_1_bus/LConn1 -- Array Connection/LConn85
  Pipe18_1/LConn2 -- H_18_1/LConn1
  Pipe18_1/RConn1 -- Pipe18_2/LConn1
  H_17_1_bus/LConn1 -- Array Connection/LConn84
  Pipe17_1/LConn2 -- H_17_1/LConn1
  H_16_2_bus/LConn1 -- Array Connection/LConn83
  Pipe16_2/LConn2 -- H_16_2/LConn1
  H_16_1_bus/LConn1 -- Array Connection/LConn82
  Pipe16_1/LConn2 -- H_16_1/LConn1
  Pipe16_1/RConn1 -- Pipe16_2/LConn1
  H_15_2_bus/LConn1 -- Array Connection/LConn81
  Pipe15_2/LConn2 -- H_15_2/LConn1
  H_15_1_bus/LConn1 -- Array Connection/LConn80
  Pipe15_1/LConn2 -- H_15_1/LConn1
  Pipe15_1/RConn1 -- Pipe15_2/LConn1
  H_14_1_bus/LConn1 -- Array Connection/LConn79
  Pipe14_1/LConn2 -- H_14_1/LConn1
  Pipe13_1/LConn1 -- Bend1_1/LConn2
  Pipe37_1/RConn1 -- fluid_out/RConn1 -- Pipe13_6/RConn1
  H_13_6_bus/LConn1 -- Array Connection/LConn78
  Pipe13_6/LConn2 -- H_13_6/LConn1
  H_13_5_bus/LConn1 -- Array Connection/LConn77
  Pipe13_5/LConn2 -- H_13_5/LConn1
  H_13_4_bus/LConn1 -- Array Connection/LConn76
  Pipe13_4/LConn2 -- H_13_4/LConn1
  H_13_3_bus/LConn1 -- Array Connection/LConn75
  Pipe13_3/LConn2 -- H_13_3/LConn1
  H_13_2_bus/LConn1 -- Array Connection/LConn74
  Pipe13_2/LConn2 -- H_13_2/LConn1
  H_13_1_bus/LConn1 -- Array Connection/LConn73
  Pipe13_1/LConn2 -- H_13_1/LConn1
  Pipe13_5/RConn1 -- Pipe13_6/LConn1
  Pipe13_4/RConn1 -- Pipe13_5/LConn1
  Pipe13_3/RConn1 -- Pipe13_4/LConn1
  Pipe13_2/RConn1 -- Pipe13_3/LConn1
  Pipe13_1/RConn1 -- Pipe13_2/LConn1
  Pipe25_1/LConn1 -- Pipe24_2/RConn1 -- Pipe12_1/LConn1
  Pipe36_2/RConn1 -- Pipe37_1/LConn1 -- Pipe12_6/RConn1
  H_12_6_bus/LConn1 -- Array Connection/LConn72
  Pipe12_6/LConn2 -- H_12_6/LConn1
  H_12_5_bus/LConn1 -- Array Connection/LConn71
  Pipe12_5/LConn2 -- H_12_5/LConn1
  H_12_4_bus/LConn1 -- Array Connection/LConn70
  Pipe12_4/LConn2 -- H_12_4/LConn1
  H_12_3_bus/LConn1 -- Array Connection/LConn69
  Pipe12_3/LConn2 -- H_12_3/LConn1
  H_12_2_bus/LConn1 -- Array Connection/LConn68
  Pipe12_2/LConn2 -- H_12_2/LConn1
  H_12_1_bus/LConn1 -- Array Connection/LConn67
  Pipe12_1/LConn2 -- H_12_1/LConn1
  Pipe12_5/RConn1 -- Pipe12_6/LConn1
  Pipe12_4/RConn1 -- Pipe12_5/LConn1
  Pipe12_3/RConn1 -- Pipe12_4/LConn1
  Pipe12_2/RConn1 -- Pipe12_3/LConn1
  Pipe12_1/RConn1 -- Pipe12_2/LConn1
  Pipe24_1/LConn1 -- Pipe23_2/RConn1 -- Pipe11_1/LConn1
  Pipe35_2/RConn1 -- Pipe36_1/LConn1 -- Pipe11_6/RConn1
  H_11_6_bus/LConn1 -- Array Connection/LConn66
  Pipe11_6/LConn2 -- H_11_6/LConn1
  H_11_5_bus/LConn1 -- Array Connection/LConn65
  Pipe11_5/LConn2 -- H_11_5/LConn1
  H_11_4_bus/LConn1 -- Array Connection/LConn64
  Pipe11_4/LConn2 -- H_11_4/LConn1
  H_11_3_bus/LConn1 -- Array Connection/LConn63
  Pipe11_3/LConn2 -- H_11_3/LConn1
  H_11_2_bus/LConn1 -- Array Connection/LConn62
  Pipe11_2/LConn2 -- H_11_2/LConn1
  H_11_1_bus/LConn1 -- Array Connection/LConn61
  Pipe11_1/LConn2 -- H_11_1/LConn1
  Pipe11_5/RConn1 -- Pipe11_6/LConn1
  Pipe11_4/RConn1 -- Pipe11_5/LConn1
  Pipe11_3/RConn1 -- Pipe11_4/LConn1
  Pipe11_2/RConn1 -- Pipe11_3/LConn1
  Pipe11_1/RConn1 -- Pipe11_2/LConn1
  Pipe23_1/LConn1 -- Pipe22_1/RConn1 -- Pipe10_1/LConn1
  Pipe34_1/RConn1 -- Pipe35_1/LConn1 -- Pipe10_6/RConn1
  H_10_6_bus/LConn1 -- Array Connection/LConn60
  Pipe10_6/LConn2 -- H_10_6/LConn1
  H_10_5_bus/LConn1 -- Array Connection/LConn59
  Pipe10_5/LConn2 -- H_10_5/LConn1
  H_10_4_bus/LConn1 -- Array Connection/LConn58
  Pipe10_4/LConn2 -- H_10_4/LConn1
  H_10_3_bus/LConn1 -- Array Connection/LConn57
  Pipe10_3/LConn2 -- H_10_3/LConn1
  H_10_2_bus/LConn1 -- Array Connection/LConn56
  Pipe10_2/LConn2 -- H_10_2/LConn1
  H_10_1_bus/LConn1 -- Array Connection/LConn55
  Pipe10_1/LConn2 -- H_10_1/LConn1
  Pipe10_5/RConn1 -- Pipe10_6/LConn1
  Pipe10_4/RConn1 -- Pipe10_5/LConn1
  Pipe10_3/RConn1 -- Pipe10_4/LConn1
  Pipe10_2/RConn1 -- Pipe10_3/LConn1
  Pipe10_1/RConn1 -- Pipe10_2/LConn1
  Pipe22_1/LConn1 -- Pipe21_2/RConn1 -- Pipe9_1/LConn1
  Pipe33_2/RConn1 -- Pipe34_1/LConn1 -- Pipe9_6/RConn1
  H_9_6_bus/LConn1 -- Array Connection/LConn54
  Pipe9_6/LConn2 -- H_9_6/LConn1
  H_9_5_bus/LConn1 -- Array Connection/LConn53
  Pipe9_5/LConn2 -- H_9_5/LConn1
  H_9_4_bus/LConn1 -- Array Connection/LConn52
  Pipe9_4/LConn2 -- H_9_4/LConn1
  H_9_3_bus/LConn1 -- Array Connection/LConn51
  Pipe9_3/LConn2 -- H_9_3/LConn1
  H_9_2_bus/LConn1 -- Array Connection/LConn50
  Pipe9_2/LConn2 -- H_9_2/LConn1
  H_9_1_bus/LConn1 -- Array Connection/LConn49
  Pipe9_1/LConn2 -- H_9_1/LConn1
  Pipe9_5/RConn1 -- Pipe9_6/LConn1
  Pipe9_4/RConn1 -- Pipe9_5/LConn1
  Pipe9_3/RConn1 -- Pipe9_4/LConn1
  Pipe9_2/RConn1 -- Pipe9_3/LConn1
  Pipe9_1/RConn1 -- Pipe9_2/LConn1
  Pipe21_1/LConn1 -- Pipe20_1/RConn1 -- Pipe8_1/LConn1
  Pipe32_1/RConn1 -- Pipe33_1/LConn1 -- Pipe8_6/RConn1
  H_8_6_bus/LConn1 -- Array Connection/LConn48
  Pipe8_6/LConn2 -- H_8_6/LConn1
  H_8_5_bus/LConn1 -- Array Connection/LConn47
  Pipe8_5/LConn2 -- H_8_5/LConn1
  H_8_4_bus/LConn1 -- Array Connection/LConn46
  Pipe8_4/LConn2 -- H_8_4/LConn1
  H_8_3_bus/LConn1 -- Array Connection/LConn45
  Pipe8_3/LConn2 -- H_8_3/LConn1
  H_8_2_bus/LConn1 -- Array Connection/LConn44
  Pipe8_2/LConn2 -- H_8_2/LConn1
  H_8_1_bus/LConn1 -- Array Connection/LConn43
  Pipe8_1/LConn2 -- H_8_1/LConn1
  Pipe8_5/RConn1 -- Pipe8_6/LConn1
  Pipe8_4/RConn1 -- Pipe8_5/LConn1
  Pipe8_3/RConn1 -- Pipe8_4/LConn1
  Pipe8_2/RConn1 -- Pipe8_3/LConn1
  Pipe8_1/RConn1 -- Pipe8_2/LConn1
  Pipe20_1/LConn1 -- Pipe19_1/RConn1 -- Pipe7_1/LConn1
  Pipe31_1/RConn1 -- Pipe32_1/LConn1 -- Pipe7_6/RConn1
  H_7_6_bus/LConn1 -- Array Connection/LConn42
  Pipe7_6/LConn2 -- H_7_6/LConn1
  H_7_5_bus/LConn1 -- Array Connection/LConn41
  Pipe7_5/LConn2 -- H_7_5/LConn1
  H_7_4_bus/LConn1 -- Array Connection/LConn40
  Pipe7_4/LConn2 -- H_7_4/LConn1
  H_7_3_bus/LConn1 -- Array Connection/LConn39
  Pipe7_3/LConn2 -- H_7_3/LConn1
  H_7_2_bus/LConn1 -- Array Connection/LConn38
  Pipe7_2/LConn2 -- H_7_2/LConn1
  H_7_1_bus/LConn1 -- Array Connection/LConn37
  Pipe7_1/LConn2 -- H_7_1/LConn1
  Pipe7_5/RConn1 -- Pipe7_6/LConn1
  Pipe7_4/RConn1 -- Pipe7_5/LConn1
  Pipe7_3/RConn1 -- Pipe7_4/LConn1
  Pipe7_2/RConn1 -- Pipe7_3/LConn1
  Pipe7_1/RConn1 -- Pipe7_2/LConn1
  Pipe19_1/LConn1 -- Pipe18_2/RConn1 -- Pipe6_1/LConn1
  Pipe30_2/RConn1 -- Pipe31_1/LConn1 -- Pipe6_6/RConn1
  H_6_6_bus/LConn1 -- Array Connection/LConn36
  Pipe6_6/LConn2 -- H_6_6/LConn1
  H_6_5_bus/LConn1 -- Array Connection/LConn35
  Pipe6_5/LConn2 -- H_6_5/LConn1
  H_6_4_bus/LConn1 -- Array Connection/LConn34
  Pipe6_4/LConn2 -- H_6_4/LConn1
  H_6_3_bus/LConn1 -- Array Connection/LConn33
  Pipe6_3/LConn2 -- H_6_3/LConn1
  H_6_2_bus/LConn1 -- Array Connection/LConn32
  Pipe6_2/LConn2 -- H_6_2/LConn1
  H_6_1_bus/LConn1 -- Array Connection/LConn31
  Pipe6_1/LConn2 -- H_6_1/LConn1
  Pipe6_5/RConn1 -- Pipe6_6/LConn1
  Pipe6_4/RConn1 -- Pipe6_5/LConn1
  Pipe6_3/RConn1 -- Pipe6_4/LConn1
  Pipe6_2/RConn1 -- Pipe6_3/LConn1
  Pipe6_1/RConn1 -- Pipe6_2/LConn1
  Pipe18_1/LConn1 -- Pipe17_1/RConn1 -- Pipe5_1/LConn1
  Pipe29_1/RConn1 -- Pipe30_1/LConn1 -- Pipe5_6/RConn1
  H_5_6_bus/LConn1 -- Array Connection/LConn30
  Pipe5_6/LConn2 -- H_5_6/LConn1
  H_5_5_bus/LConn1 -- Array Connection/LConn29
  Pipe5_5/LConn2 -- H_5_5/LConn1
  H_5_4_bus/LConn1 -- Array Connection/LConn28
  Pipe5_4/LConn2 -- H_5_4/LConn1
  H_5_3_bus/LConn1 -- Array Connection/LConn27
  Pipe5_3/LConn2 -- H_5_3/LConn1
  H_5_2_bus/LConn1 -- Array Connection/LConn26
  Pipe5_2/LConn2 -- H_5_2/LConn1
  H_5_1_bus/LConn1 -- Array Connection/LConn25
  Pipe5_1/LConn2 -- H_5_1/LConn1
  Pipe5_5/RConn1 -- Pipe5_6/LConn1
  Pipe5_4/RConn1 -- Pipe5_5/LConn1
  Pipe5_3/RConn1 -- Pipe5_4/LConn1
  Pipe5_2/RConn1 -- Pipe5_3/LConn1
  Pipe5_1/RConn1 -- Pipe5_2/LConn1
  Pipe17_1/LConn1 -- Pipe16_2/RConn1 -- Pipe4_1/LConn1
  Pipe28_2/RConn1 -- Pipe29_1/LConn1 -- Pipe4_6/RConn1
  H_4_6_bus/LConn1 -- Array Connection/LConn24
  Pipe4_6/LConn2 -- H_4_6/LConn1
  H_4_5_bus/LConn1 -- Array Connection/LConn23
  Pipe4_5/LConn2 -- H_4_5/LConn1
  H_4_4_bus/LConn1 -- Array Connection/LConn22
  Pipe4_4/LConn2 -- H_4_4/LConn1
  H_4_3_bus/LConn1 -- Array Connection/LConn21
  Pipe4_3/LConn2 -- H_4_3/LConn1
  H_4_2_bus/LConn1 -- Array Connection/LConn20
  Pipe4_2/LConn2 -- H_4_2/LConn1
  H_4_1_bus/LConn1 -- Array Connection/LConn19
  Pipe4_1/LConn2 -- H_4_1/LConn1
  Pipe4_5/RConn1 -- Pipe4_6/LConn1
  Pipe4_4/RConn1 -- Pipe4_5/LConn1
  Pipe4_3/RConn1 -- Pipe4_4/LConn1
  Pipe4_2/RConn1 -- Pipe4_3/LConn1
  Pipe4_1/RConn1 -- Pipe4_2/LConn1
  Pipe16_1/LConn1 -- Pipe15_2/RConn1 -- Pipe3_1/LConn1
  Pipe27_2/RConn1 -- Pipe28_1/LConn1 -- Pipe3_6/RConn1
  H_3_6_bus/LConn1 -- Array Connection/LConn18
  Pipe3_6/LConn2 -- H_3_6/LConn1
  H_3_5_bus/LConn1 -- Array Connection/LConn17
  Pipe3_5/LConn2 -- H_3_5/LConn1
  H_3_4_bus/LConn1 -- Array Connection/LConn16
  Pipe3_4/LConn2 -- H_3_4/LConn1
  H_3_3_bus/LConn1 -- Array Connection/LConn15
  Pipe3_3/LConn2 -- H_3_3/LConn1
  H_3_2_bus/LConn1 -- Array Connection/LConn14
  Pipe3_2/LConn2 -- H_3_2/LConn1
  H_3_1_bus/LConn1 -- Array Connection/LConn13
  Pipe3_1/LConn2 -- H_3_1/LConn1
  Pipe3_5/RConn1 -- Pipe3_6/LConn1
  Pipe3_4/RConn1 -- Pipe3_5/LConn1
  Pipe3_3/RConn1 -- Pipe3_4/LConn1
  Pipe3_2/RConn1 -- Pipe3_3/LConn1
  Pipe3_1/RConn1 -- Pipe3_2/LConn1
  Pipe15_1/LConn1 -- Pipe14_1/RConn1 -- Pipe2_1/LConn1
  Pipe26_1/RConn1 -- Pipe27_1/LConn1 -- Pipe2_6/RConn1
  H_2_6_bus/LConn1 -- Array Connection/LConn12
  Pipe2_6/LConn2 -- H_2_6/LConn1
  H_2_5_bus/LConn1 -- Array Connection/LConn11
  Pipe2_5/LConn2 -- H_2_5/LConn1
  H_2_4_bus/LConn1 -- Array Connection/LConn10
  Pipe2_4/LConn2 -- H_2_4/LConn1
  H_2_3_bus/LConn1 -- Array Connection/LConn9
  Pipe2_3/LConn2 -- H_2_3/LConn1
  H_2_2_bus/LConn1 -- Array Connection/LConn8
  Pipe2_2/LConn2 -- H_2_2/LConn1
  H_2_1_bus/LConn1 -- Array Connection/LConn7
  Pipe2_1/LConn2 -- H_2_1/LConn1
  Pipe2_5/RConn1 -- Pipe2_6/LConn1
  Pipe2_4/RConn1 -- Pipe2_5/LConn1
  Pipe2_3/RConn1 -- Pipe2_4/LConn1
  Pipe2_2/RConn1 -- Pipe2_3/LConn1
  Pipe2_1/RConn1 -- Pipe2_2/LConn1
  Pipe14_1/LConn1 -- fluid_in/RConn1 -- Pipe1_1/LConn1
  Pipe1_6/RConn1 -- Bend2_1/LConn1
  H_1_6_bus/LConn1 -- Array Connection/LConn6
  Pipe1_6/LConn2 -- H_1_6/LConn1
  H_1_5_bus/LConn1 -- Array Connection/LConn5
  Pipe1_5/LConn2 -- H_1_5/LConn1
  H_1_4_bus/LConn1 -- Array Connection/LConn4
  Pipe1_4/LConn2 -- H_1_4/LConn1
  H_1_3_bus/LConn1 -- Array Connection/LConn3
  Pipe1_3/LConn2 -- H_1_3/LConn1
  H_1_2_bus/LConn1 -- Array Connection/LConn2
  Pipe1_2/LConn2 -- H_1_2/LConn1
  H_1_1_bus/LConn1 -- Array Connection/LConn1
  Pipe1_1/LConn2 -- H_1_1/LConn1
  Pipe1_5/RConn1 -- Pipe1_6/LConn1
  Pipe1_4/RConn1 -- Pipe1_5/LConn1
  Pipe1_3/RConn1 -- Pipe1_4/LConn1
  Pipe1_2/RConn1 -- Pipe1_3/LConn1
  Pipe1_1/RConn1 -- Pipe1_2/LConn1
